simulink model "SWC_HALIN_CDD_type"  (R2021b)
settings: Solver=FixedStepDiscrete  StartTime=0.0  StopTime=10.0  FixedStep=0.005  RelTol=1e-3
values from neighbouring files (symbols this model uses):
  C_TASK_5MS_S = (	C_TICK_TIME_S      	)    [vcu_local_hdr.m]    (also in vcu_local_hdrTA2.m)
  DIDLen_APSFunConfig = uint16(16)    [vcu_local_hdr.m]
  DIDLen_AutoLock = uint16(1)    [vcu_local_hdr.m]
  DIDLen_AutoWipHSpdEN = uint16(1)    [vcu_local_hdr.m]
  DIDLen_DKCKey = uint16(8)    [vcu_local_hdr.m]
  DIDLen_DRLDis = uint16(1)    [vcu_local_hdr.m]
  DIDLen_DynoMode = uint16(1)    [vcu_local_hdr.m]
  DIDLen_FMHTimer = uint16(1)    [vcu_local_hdr.m]
  DIDLen_TireSize = uint16(16)    [vcu_local_hdr.m]
  DIDLen_TurnLampFLThreCurr = uint16(1)    [vcu_local_hdr.m]
  DIDLen_TurnLampFRThreCurr = uint16(1)    [vcu_local_hdr.m]
  DIDLen_TurnLampRLThreCurr = uint16(1)    [vcu_local_hdr.m]
  DIDLen_TurnLampRRThreCurr = uint16(1)    [vcu_local_hdr.m]
  DIDLen_USSConfig = uint16(16)    [vcu_local_hdr.m]
  DIDLen_WipRLSCmdCutFilter = uint16(1)    [vcu_local_hdr.m]
  DIDLen_WipRLSCmdHoldFilter = uint16(1)    [vcu_local_hdr.m]
  DIDLen_XWDMode = uint16(1)    [vcu_local_hdr.m]
  DIDNum_APSFunConfig = uint16(0x0903)    [vcu_local_hdr.m]
  DIDNum_AutoLock = uint16(0x0306)    [vcu_local_hdr.m]
  DIDNum_AutoWipHSpdEN = uint16(0x0308)    [vcu_local_hdr.m]
  DIDNum_DKCKey = uint16(0x0202)    [vcu_local_hdr.m]
  DIDNum_DRLDis = uint16(0x0307)    [vcu_local_hdr.m]
  DIDNum_DynoMode = uint16(0x0203)    [vcu_local_hdr.m]
  DIDNum_FMHTimer = uint16(0x0305)    [vcu_local_hdr.m]
  DIDNum_TireSize = uint16(0x0902)    [vcu_local_hdr.m]
  DIDNum_TurnLampFLThreCurr = uint16(0x0303)    [vcu_local_hdr.m]
  DIDNum_TurnLampFRThreCurr = uint16(0x0301)    [vcu_local_hdr.m]
  DIDNum_TurnLampRLThreCurr = uint16(0x0304)    [vcu_local_hdr.m]
  DIDNum_TurnLampRRThreCurr = uint16(0x0302)    [vcu_local_hdr.m]
  DIDNum_USSConfig = uint16(0x0901)    [vcu_local_hdr.m]
  DIDNum_WipRLSCmdCutFilter = uint16(0x030A)    [vcu_local_hdr.m]
  DIDNum_WipRLSCmdHoldFilter = uint16(0x0309)    [vcu_local_hdr.m]
  DIDNum_XWDMode = uint16(0x0201)    [vcu_local_hdr.m]
  ENUM_DRIVETRAIN_AWD = uint8(  2  )    [vcu_local_hdr.m]
  ENUM_DRIVETRAIN_FWD = uint8(  1  )    [vcu_local_hdr.m]
  ENUM_DRIVETRAIN_RWD = uint8(  0  )    [vcu_local_hdr.m]
  ENUM_REGENLEVEL_LV1 = uint8(  1  )    [vcu_local_hdr.m]
  ENUM_REGENLEVEL_LV2 = uint8(  2  )    [vcu_local_hdr.m]
  ENUM_REGENLEVEL_LV3 = uint8(  3  )    [vcu_local_hdr.m]
  ENUM_REGENLEVEL_LV4 = uint8(  4  )    [vcu_local_hdr.m]
  ENUM_REGENLEVEL_LV5 = uint8(  5  )    [vcu_local_hdr.m]
  ENUM_REGENLEVEL_OPD = uint8(  6  )    [vcu_local_hdr.m]
  ENUM_TPMSSTA_FAT = uint8(  8  )    [vcu_local_hdr.m]
  ENUM_TPMSSTA_LOWBATTERY = uint8(  2  )    [vcu_local_hdr.m]
  ENUM_TPMSSTA_TRIGGER = uint8(  4  )    [vcu_local_hdr.m]
  FALSE = boolean( 0 )    [vcu_local_hdr.m]    (also in vcu_local_hdrTA2.m)
  ONE_INT = uint8(1)    [vcu_local_hdr.m]    (also in vcu_local_hdrTA2.m)
  TRUE = boolean( 1 )    [vcu_local_hdr.m]    (also in vcu_local_hdrTA2.m)
  ZERO_FLOAT = single(0)    [vcu_local_hdr.m]    (also in vcu_local_hdrTA2.m)
  ZERO_INT = uint8(0)    [vcu_local_hdr.m]    (also in vcu_local_hdrTA2.m)
undefined symbols (not defined in the file or in its folder): KHAL_CANBusOffDebounce_s, KHAL_DefaultRegenMode_enum, KHAL_DKCDecryptEnable_flg_ovrdflg, KHAL_DKCDecryptEnable_flg_ovrdval, KHAL_RandomNumberY1_enum, KHAL_RandomNumberY2_enum, KHAL_RandomNumberY_ovrdflg, KHAL_TPMSRESBUTT_flg_ovrdflg, KHAL_TPMSRESBUTT_flg_ovrdval, KINP_ReadVinCode_flg, R_NVMReadCDD_Inner_NVM_ReadOperation
libraries: simulink x112, hcu_lib x23, hdlsllib x8
(part 4 of 7)

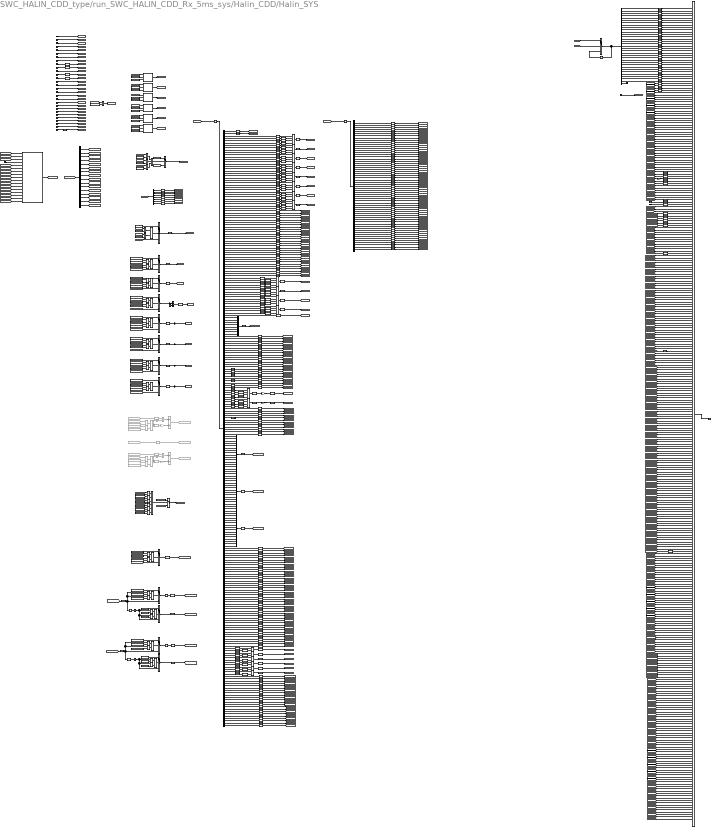
== system SWC_HALIN_CDD_type/run_SWC_HALIN_CDD_Rx_5ms_sys/Halin_CDD/Halin_SYS ==
  note: DID XWD
  note: DID VCUKey
  note: DID BCM
  note: DID APS
  note: CAN bus off debounce
  GetSWID_status : Inport
  GetSWID_data : Inport  Port=2
  VHAL_AnyNMID_flg : Inport  Port=3
  VHAL_CurrentNmState_enum : Inport  Port=4
  VHAL_PwrReq_OTA_enum : Inport  Port=5
  VHAL_AllowMovThd_OTA_enum : Inport  Port=6
  VHAL_EvccAplusPwrUpReq_flg : Inport  Port=7
  VHAL_AcoreReadyToSlp_flg : Inport  Port=8
  VHAL_DidXWDSta_flg : Inport  Port=9
  VHAL_DidXWDData_enum : Inport  Port=10
  HAL_NvmReadData_raw : Inport  Port=11
  VHAL_DIDVCUKeyReadSta_flg : Inport  Port=12
  VHAL_GetDIDVCUKey_enum : Inport  Port=13
  VHAL_NvmProtectSta_flg : Inport  Port=14
  VHAL_AuxBattVolmV_100mV : Inport  Port=15
  VHAL_Pedal1Ref5V_raw : Inport  Port=16
  VHAL_Pedal2Ref5V_raw : Inport  Port=17
  VHAL_NetworkReqCalled_flg : Inport  Port=18
  VHAL_PmicBootReason_enum : Inport  Port=19
  VHAL_WisrBootReason_raw32 : Inport  Port=20
  BHAL_DIDGetData_raw : Inport  Port=21
  VHAL_AcoreRebootCmd_raw : Inport  Port=22
  VHAL_CAN1BusOff_raw : Inport  Port=23
  VHAL_CAN2BusOff_raw : Inport  Port=24
  VHAL_CAN3BusOff_raw : Inport  Port=25
  VHAL_CAN4BusOff_raw : Inport  Port=26
  VHAL_CAN5BusOff_raw : Inport  Port=27
  VHAL_CAN6BusOff_raw : Inport  Port=28
  u8_TPMSSensorIDRegSta : Inport  Port=29
  VHAL_ResetPedalZeroPosReq_raw : Inport  Port=30
  VHAL_PmicBootPath_raw32 : Inport  Port=31
  AND : Logic  Inputs=6  AllPortsSameDT=off  OutDataTypeStr=boolean
  Add1 : Sum
  Bit Shift : hdlsllib/Logic and Bit Operations/Bit Shift  mode=Shift Right Logical  N=1
  Bit Shift1 : hdlsllib/Logic and Bit Operations/Bit Shift  mode=Shift Right Logical  N=1
  Bitwise AND : simulink/Logic and Bit Operations/Bitwise Operator  logicop=AND  UseBitMask=on  BitMask=bin2dec('1')  BitMaskRealWorld=Stored Integer
  Bitwise AND1 : simulink/Logic and Bit Operations/Bitwise Operator  logicop=AND  UseBitMask=on  BitMask=bin2dec('1111111')  BitMaskRealWorld=Stored Integer
  Bitwise AND2 : simulink/Logic and Bit Operations/Bitwise Operator  logicop=AND  UseBitMask=on  BitMask=bin2dec('1')  BitMaskRealWorld=Stored Integer
  Bitwise AND3 : simulink/Logic and Bit Operations/Bitwise Operator  logicop=AND  UseBitMask=on  BitMask=bin2dec('1111111')  BitMaskRealWorld=Stored Integer
  Bitwise OR{1..14} (14 alike) : simulink/Logic and Bit Operations/Bitwise Operator  logicop=OR  UseBitMask=off  NumInputPorts=4  BitMask=bin2dec('00000000000000000000')  BitMaskRealWorld=Stored Integer
  Bitwise OR{15..20} (6 alike) : simulink/Logic and Bit Operations/Bitwise Operator  logicop=OR  UseBitMask=off  NumInputPorts=2  BitMask=bin2dec('00000000000000000000')  BitMaskRealWorld=Stored Integer
  Bus Creator : BusCreator  Inputs=349  OutDataTypeStr=Bus: BHAL_SYS_outputs  NonVirtualBus=on
  Bus Selector : BusSelector  OutputSignals=VHAL_DIDGetXWDMode_raw8,VHAL_DIDGetDKCKey_raw8,VHAL_DIDGetDynoMode_raw8,VHAL_DIDGetTurnLampFRThreCurr_raw8,VHAL_DIDGetTurnLampRRThreCurr_raw8,VHAL_DIDGetTurnLampFLThreCurr_raw8,VHAL_DIDGetTurnLampRLThreCurr_raw8,VHAL_DIDGetFMHTimer_raw8,VHAL_DIDGetAutoLock_raw8,VHAL_DIDGetDRLDis_raw8,VHAL_DIDGetAutoWipHSpdEN_raw8,VHAL_DIDGetWipRLSCmdHoldFilter_raw8,VHAL_DIDGetWipRLSCmdCutFilter_raw8,VHAL_DIDGetUSSConfig_raw8,VHAL_DIDGetTireSize_raw8,VHAL_DIDGetAPSFunConfig_raw8
  Constant{,2..3,10..11,14..15,17,23,26,33,43,47,50,53} (15 alike) : Constant  Value=ZERO_INT
  Constant{1,22,25,41} (4 alike) : Constant  Value=ONE_INT
  Constant12 : Constant  Value=10  OutDataTypeStr=uint8
  Constant{9,13,19..20,28,51,54} (7 alike) : Constant  Value=254  OutDataTypeStr=uint8
  Constant16 : Constant  Value=40  OutDataTypeStr=uint8
  Constant18 : Constant  Value=40  OutDataTypeStr=uint8
  Constant{21,24,42,52,55} (5 alike) : Constant  Value=ZERO_INT  OutDataTypeStr=uint8
  Constant27 : Constant  Value=6  OutDataTypeStr=uint8
  Constant29 : Constant  Commented=on  Value=ONE_INT
  Constant30 : Constant  Commented=on  Value=ZERO_INT
  Constant31 : Constant  Commented=on  Value=ONE_INT
  Constant32 : Constant  Commented=on  Value=ZERO_INT
  Constant34 : Constant  Value=ENUM_REGENLEVEL_LV1
  Constant35 : Constant  Value=ENUM_REGENLEVEL_LV2
  Constant36 : Constant  Value=ENUM_REGENLEVEL_LV3
  Constant37 : Constant  Value=ENUM_REGENLEVEL_LV4
  Constant38 : Constant  Value=ENUM_REGENLEVEL_LV5
  Constant39 : Constant  Value=ENUM_REGENLEVEL_OPD
  Constant4 : Constant  Value=10  OutDataTypeStr=uint8
  Constant40 : Constant  Value=KHAL_DefaultRegenMode_enum
  Constant44 : Constant  Value=126  OutDataTypeStr=uint8
  Constant45 : Constant  Value=10
  Constant46 : Constant  Value=2  OutDataTypeStr=uint8
  Constant48 : Constant  Value=126  OutDataTypeStr=uint8
  Constant49 : Constant  Value=5  OutDataTypeStr=uint8
  Constant5 : Constant  Value=ENUM_DRIVETRAIN_FWD
  Constant{56,58,60,62,64,66} (6 alike) : Constant  Value=C_TASK_5MS_S  OutDataTypeStr=single
  Constant{57,59,61,63,65,67} (6 alike) : Constant  Value=KHAL_CANBusOffDebounce_s  OutDataTypeStr=single
  Constant6 : Constant  Value=ENUM_DRIVETRAIN_RWD
  Constant7 : Constant  Value=ENUM_DRIVETRAIN_AWD
  Constant8 : Constant  Value=ENUM_DRIVETRAIN_RWD
  DIDGet_List : Subsystem
  Data Type Conversion{,3..30,33..44,49..55,98..104,106..107,109,112..128,130..135,139..141,143,164,187,190..195,208..210,212..253,255,273..282,285..286,288..293,296..297,299..358,360..363,814..822} (232 alike) : DataTypeConversion  OutDataTypeStr=uint8
  Data Type Conversion{1..2,31..32,45..48,56..57,105,108,110..111,129,136..138,142,180..185,188..189,200..201,211,283..284,287,294,298,359,823} (37 alike) : DataTypeConversion  OutDataTypeStr=boolean
  Data Type Conversion{58..97,144..163,169..178,186,295} (72 alike) : DataTypeConversion  OutDataTypeStr=uint32
  Data Type Conversion{165..166,168,179,196..199,202} (9 alike) : DataTypeConversion  OutDataTypeStr=single
  Data Type Conversion{167,254,256..272} (19 alike) : DataTypeConversion  OutDataTypeStr=uint16
  Data Type Conversion{203..207} (5 alike) : DataTypeConversion  Commented=on  OutDataTypeStr=uint8
  Demux : Demux  Outputs=33
  Demux1 : Demux  Outputs=256
  Demux2 : Demux  Outputs=8
  Demux3 : Demux  Outputs=61
  Equal{1..5,24..25,28..31} (11 alike) : RelationalOperator  Operator=~=  OutDataTypeStr=boolean  RndMeth=Simplest
  Equal{6,8,10,12,14,16,18,26,32,34,36,38} (12 alike) : RelationalOperator  Operator=>  OutDataTypeStr=boolean  RndMeth=Simplest
  Equal{7,9,11,13,15,17,19,27,33,35,37,39} (12 alike) : RelationalOperator  Operator=<  OutDataTypeStr=boolean  RndMeth=Simplest
  Equal{20..23} (4 alike) : RelationalOperator  Commented=on  Operator=~=  OutDataTypeStr=boolean  RndMeth=Simplest
  FlashAPMDoorControlSta : Subsystem
  FlashCountAlarm_Verify : Subsystem
  FlashFuelDoorPos_Verify : Subsystem
  FlashIVIPTGUSStaSW_Verify : Subsystem
  FlashMFRDNBrightReq_Verify : Subsystem
  FlashMFSWTri_Verify : Subsystem
  FlashMirrorFlodPos_Verify : Subsystem
  FlashWiperFixMode_Verify : Subsystem
  From113 : From  Commented=on  GotoTag=VHAL_DIDGetUSSConfig_raw8
  From114 : From  Commented=on  GotoTag=VHAL_DIDGetTireSize_raw8
  From115 : From  Commented=on  GotoTag=VHAL_DIDGetAPSFunConfig_raw8
  From116 : From  Commented=on  GotoTag=VHAL_DIDGetUSSConfig_raw8
  From117 : From  Commented=on  GotoTag=VHAL_DIDGetUSSConfig_raw8
  From118 : From  Commented=on  GotoTag=VHAL_DIDGetAPSFunConfig_raw8
  From119 : From  Commented=on  GotoTag=VHAL_DIDGetAPSFunConfig_raw8
  Gain2 : Gain  Gain=100
  Gain3 : Gain  Gain=5
  Gain{4..7} (4 alike) : Gain  Gain=10
  Gain8 : Gain  Commented=on  Gain=0xFF  OutDataTypeStr=uint8
  Gain9 : Gain  Commented=on  Gain=0xFF  OutDataTypeStr=uint8
  Goto140 : Goto  Commented=on  GotoTag=VHAL_USSConfig_raw8
  Goto142 : Goto  Commented=on  GotoTag=VHAL_TireSize_raw8
  Goto143 : Goto  Commented=on  GotoTag=VHAL_APSFunConfig_raw8
  Ground : Ground
  Ground1 : Ground
  LatchedFlg{,1..5} (6 alike) : hcu_lib/Basic_Blocks/LatchedFlg
  Logical Operator : Logic  Inputs=3  AllPortsSameDT=off  OutDataTypeStr=boolean
  Logical Operator1 : Logic  AllPortsSameDT=off  OutDataTypeStr=boolean
  Logical Operator{2..13} (12 alike) : Logic  Operator=OR  AllPortsSameDT=off  OutDataTypeStr=boolean
  Multiply1 : Gain  Gain=1/10000
  Multiply2 : Gain  Gain=1/10000
  Mux : Mux  Inputs=8
  Mux1 : Mux  Inputs=16
  Mux2 : Mux  Inputs=16
  Mux3 : Mux  Inputs=16
  NOT : Logic  Commented=on  Operator=NOT  AllPortsSameDT=off  OutDataTypeStr=boolean
  NOT1 : Logic  Commented=on  Operator=NOT  AllPortsSameDT=off  OutDataTypeStr=boolean
  NotEqual : RelationalOperator  Operator=~=  OutDataTypeStr=boolean  RndMeth=Simplest
  OR : Logic  Commented=on  AllPortsSameDT=off  OutDataTypeStr=boolean
  OR1 : Logic  Commented=on  AllPortsSameDT=off  OutDataTypeStr=boolean
  Product : Product  Commented=on
  Product1 : Product  Commented=on
  Selector1 : Selector  InputPortWidth=1024  IndexOptions=Index vector (dialog)  Indices=[1:256]  OutputSizes=1
  Selector2 : Selector  InputPortWidth=1024  IndexOptions=Index vector (dialog)  Indices=[257:317]  OutputSizes=1
  Shift Arithmetic{1,6,9,12,16,21,25,28..29,32,35..37,40,43..48} (20 alike) : ArithShift  BitShiftNumber=8  BitShiftDirection=Left
  Shift Arithmetic{2..3,7,10,13..14,17..18,22,26,30,33,38,41} (14 alike) : ArithShift  BitShiftNumber=16  BitShiftDirection=Left
  Shift Arithmetic{4..5,8,11,15,19..20,23..24,27,31,34,39,42} (14 alike) : ArithShift  BitShiftNumber=24  BitShiftDirection=Left
  Sum : Sum  Commented=on
  Sum1 : Sum  Commented=on
  Switch{,1..15} (16 alike) : Switch  Criteria=u2 ~= 0
  Terminator3 : Terminator
  Unit Delay1 : UnitDelay  SampleTime=-1  HasFrameUpgradeWarning=on
  BHAL_SYS_outputs : Outport  OutDataTypeStr=Bus:BHAL_SYS_outputs
  wires:
  Data Type Conversion49/1 -> [VHAL_RFWheelPSW_raw8]  "VHAL_RFWheelPSW_raw8"
  Demux1/36 -> Data Type Conversion46/1
  Data Type Conversion91/1 -> Shift Arithmetic28/1
  Shift Arithmetic29/1 -> Bitwise OR5/2
  Shift Arithmetic14/1 -> Bitwise OR7/3
  Data Type Conversion73/1 -> Bitwise OR7/1
  Demux/1 -> Data Type Conversion/1
  Data Type Conversion86/1 -> Bitwise OR10/1
  Demux1/39 -> Data Type Conversion51/1
  Demux1/23 -> Data Type Conversion82/1
  Data Type Conversion71/1 -> Shift Arithmetic33/1
  Data Type Conversion48/1 -> [VHAL_RRSensorFail_flg]  "VHAL_RRSensorFail_flg"
  Data Type Conversion11/1 -> Bus Creator/9  "VHAL_Minor2_cnt"
  Data Type Conversion90/1 -> Bitwise OR11/1
  Shift Arithmetic18/1 -> Bitwise OR11/3
  [VHAL_EvccAplusPwrUpReq_flg] -> Data Type Conversion32/1
  Demux1/31 -> Data Type Conversion90/1
  Shift Arithmetic26/1 -> Bitwise OR10/3
  Shift Arithmetic32/1 -> Bitwise OR6/2
  Shift Arithmetic15/1 -> Bitwise OR7/4
  Demux1/30 -> Data Type Conversion89/1
  Data Type Conversion16/1 -> Bus Creator/14  "VHAL_Variation_cnt"
  Data Type Conversion53/1 -> [VHAL_RFPindi_enum]  "VHAL_RFPindi_enum"
  Data Type Conversion95/1 -> [VHAL_FlashRFID_raw]  "VHAL_FlashRFID_raw"
  Demux1/7 -> Data Type Conversion65/1
  Ground/1 -> [VHAL_ReadFlashCorrect_flg]  "VHAL_ReadFlashCorrect_flg"
  Data Type Conversion92/1 -> Shift Arithmetic18/1
  Shift Arithmetic17/1 -> Bitwise OR8/3
  Shift Arithmetic16/1 -> Bitwise OR8/2
  Data Type Conversion54/1 -> [VHAL_FlashAntitheft_enum]  "VHAL_FlashAntitheft_enum"
  Shift Arithmetic22/1 -> Bitwise OR9/3
  Demux1/35 -> Data Type Conversion45/1
  Data Type Conversion78/1 -> [VHAL_FlashChkRFID_raw]  "VHAL_FlashChkRFID_raw"
  Shift Arithmetic21/1 -> Bitwise OR9/2
  Demux1/43 -> Data Type Conversion36/1
  Demux1/25 -> Data Type Conversion84/1
  Demux1/44 -> Data Type Conversion53/1
  Bus Creator/1 -> BHAL_SYS_outputs/1
  Demux1/45 -> Data Type Conversion35/1
  Demux1/14 -> Data Type Conversion72/1
  Demux1/29 -> Data Type Conversion88/1
  Demux1/24 -> Data Type Conversion83/1
  Data Type Conversion35/1 -> [VHAL_LRPindi_enum]  "VHAL_LRPindi_enum"
  Demux1/50 -> Data Type Conversion41/1
  GetSWID_status/1 -> [SYSOut]
  Data Type Conversion37/1 -> [VHAL_RRPindi_enum]  "VHAL_RRPindi_enum"
  Demux1/27 -> Data Type Conversion86/1
  Demux1/6 -> Data Type Conversion64/1
  Demux1/3 -> Data Type Conversion59/1
  Data Type Conversion41/1 -> [VHAL_RRP20_raw8]  "VHAL_RRP20_raw8"
  Constant8/1 -> Switch3/1
  Data Type Conversion70/1 -> Shift Arithmetic32/1
  [VHAL_DIDGetXWDMode_raw8] -> Equal1/1
  Data Type Conversion64/1 -> Shift Arithmetic24/1
  Demux1/9 -> Data Type Conversion67/1
  Shift Arithmetic30/1 -> Bitwise OR5/3
  Bitwise OR10/1 -> Data Type Conversion96/1
  Equal2/1 -> Logical Operator/2
  Equal1/1 -> Logical Operator/1
  Switch3/1 -> [VHAL_DrivetrainSelect_enum]  "VHAL_DrivetrainSelect_enum"
  Data Type Conversion45/1 -> [VHAL_LFSensorFail_flg]  "VHAL_LFSensorFail_flg"
  Data Type Conversion6/1 -> Bus Creator/4  "VHAL_ECU1_cnt"
  Demux/8 -> Data Type Conversion10/1
  Demux1/32 -> Data Type Conversion91/1
  Switch1/1 -> Demux/1, Unit Delay1/1
  Demux/3 -> Data Type Conversion5/1
  Data Type Conversion14/1 -> Bus Creator/12  "VHAL_Country1_cnt"
  Data Type Conversion13/1 -> Bus Creator/11  "VHAL_Patch2_cnt"
  Demux1/46 -> Data Type Conversion37/1
  Demux/11 -> Data Type Conversion13/1
  Demux/14 -> Data Type Conversion16/1
  Data Type Conversion8/1 -> Bus Creator/6  "VHAL_Major1_cnt"
  Data Type Conversion9/1 -> Bus Creator/7  "VHAL_Major2_cnt"
  Demux/13 -> Data Type Conversion15/1
  Shift Arithmetic19/1 -> Bitwise OR11/4
  Demux1/2 -> Data Type Conversion55/1
  Data Type Conversion108/1 -> [VHAL_DIDVCUKeyReadSta_flg]  "VHAL_DIDVCUKeyReadSta_flg"
  Data Type Conversion38/1 -> [VHAL_RFP20_raw8]  "VHAL_RFP20_raw8"
  [VHAL_AcoreReadyToSlp_flg] -> Data Type Conversion1/1
  Demux2/2 -> Data Type Conversion113/1
  Data Type Conversion74/1 -> Shift Arithmetic35/1
  Demux2/5 -> Data Type Conversion116/1
  [VHAL_DIDGetXWDMode_raw8] -> Equal3/1
  Data Type Conversion119/1 -> [VHAL_RandomnumberY_raw8]  "VHAL_RandomnumberY_raw8"
  Demux2/6 -> Data Type Conversion117/1
  Data Type Conversion117/1 -> [VHAL_RandomnumberY_raw6]  "VHAL_RandomnumberY_raw6"
  Demux/9 -> Data Type Conversion11/1
  Data Type Conversion60/1 -> Shift Arithmetic16/1
  Demux1/21 -> Data Type Conversion61/1
  Data Type Conversion114/1 -> [VHAL_RandomnumberY_raw3]  "VHAL_RandomnumberY_raw3"
  Data Type Conversion7/1 -> Bus Creator/5  "VHAL_ECU2_cnt"
  Data Type Conversion116/1 -> [VHAL_RandomnumberY_raw5]  "VHAL_RandomnumberY_raw5"
  Demux2/3 -> Data Type Conversion114/1
  Data Type Conversion115/1 -> [VHAL_RandomnumberY_raw4]  "VHAL_RandomnumberY_raw4"
  Shift Arithmetic25/1 -> Bitwise OR10/2
  Data Type Conversion79/1 -> [VHAL_FlashChkLRID_raw]  "VHAL_FlashChkLRID_raw"
  Data Type Conversion81/1 -> Shift Arithmetic20/1
  Demux/10 -> Data Type Conversion12/1
  Data Type Conversion113/1 -> [VHAL_RandomnumberY_raw2]  "VHAL_RandomnumberY_raw2"
  Data Type Conversion12/1 -> Bus Creator/10  "VHAL_Patch1_cnt"
  Shift Arithmetic20/1 -> Bitwise OR8/4
  Demux1/11 -> Data Type Conversion69/1
  Data Type Conversion10/1 -> Bus Creator/8  "VHAL_Minor1_cnt"
  Data Type Conversion84/1 -> Shift Arithmetic22/1
  Demux1/62 -> Data Type Conversion106/1
  Data Type Conversion94/1 -> [VHAL_FlashLFID_raw]  "VHAL_FlashLFID_raw"
  Demux1/48 -> Data Type Conversion38/1
  Data Type Conversion98/1 -> [VHAL_RFWheelTemp_C]  "VHAL_RFWheelTemp_C"
  Shift Arithmetic12/1 -> Bitwise OR4/2
  Data Type Conversion83/1 -> Shift Arithmetic21/1
  Demux1/49 -> Data Type Conversion39/1
  Demux1/13 -> Data Type Conversion71/1
  Data Type Conversion69/1 -> Bitwise OR6/1
  Demux1/61 -> Data Type Conversion105/1
  Demux1/60 -> Data Type Conversion103/1
  Data Type Conversion104/1 -> [VHAL_Flashchkdatavalid_enum]  "VHAL_Flashchkdatavalid_enum"
  Demux1/59 -> Data Type Conversion104/1
  Bitwise OR7/1 -> Data Type Conversion80/1
  Data Type Conversion103/1 -> [VHAL_Flashdatavalid_enum]  "VHAL_Flashdatavalid_enum"
  Shift Arithmetic23/1 -> Bitwise OR9/4
  Demux1/58 -> Data Type Conversion101/1
  Demux1/20 -> Data Type Conversion60/1
  Data Type Conversion99/1 -> [VHAL_LRWheelTemp_C]  "VHAL_LRWheelTemp_C"
  Demux1/54 -> Data Type Conversion44/1
  Demux/12 -> Data Type Conversion14/1
  Data Type Conversion82/1 -> Bitwise OR9/1
  Demux1/53 -> Data Type Conversion42/1
  Demux1/17 -> Data Type Conversion75/1
  Data Type Conversion96/1 -> [VHAL_FlashLRID_raw]  "VHAL_FlashLRID_raw"
  Demux1/8 -> Data Type Conversion66/1
  Demux1/37 -> Data Type Conversion47/1
  Demux1/34 -> Data Type Conversion93/1
  Demux1/10 -> Data Type Conversion68/1
  Data Type Conversion66/1 -> Shift Arithmetic29/1
  Shift Arithmetic24/1 -> Bitwise OR4/4
  Data Type Conversion15/1 -> Bus Creator/13  "VHAL_Country2_cnt"
  Data Type Conversion50/1 -> [VHAL_LRWheelPSW_raw8]  "VHAL_LRWheelPSW_raw8"
  Data Type Conversion61/1 -> Shift Arithmetic17/1
  Demux/5 -> Data Type Conversion7/1
  Bitwise OR9/1 -> Data Type Conversion95/1
  Data Type Conversion40/1 -> [VHAL_LFP20_raw8]  "VHAL_LFP20_raw8"
  Data Type Conversion112/1 -> [VHAL_RandomnumberY_raw1]  "VHAL_RandomnumberY_raw1"
  Data Type Conversion46/1 -> [VHAL_RFSensorFail_flg]  "VHAL_RFSensorFail_flg"
  Data Type Conversion88/1 -> Shift Arithmetic26/1
  Data Type Conversion67/1 -> Shift Arithmetic30/1
  Data Type Conversion87/1 -> Shift Arithmetic25/1
  Demux1/1 -> Data Type Conversion54/1
  Data Type Conversion127/1 -> [VHAL_FlashAirIntenZone1M_enum]  "VHAL_FlashAirIntenZone1M_enum"
  Demux1/33 -> Data Type Conversion92/1
  Data Type Conversion106/1 -> [VHAL_unlearnSfailvalid_enum]  "VHAL_unlearnSfailvalid_enum"
  Demux1/52 -> Data Type Conversion102/1
  Demux2/1 -> Data Type Conversion112/1
  Data Type Conversion63/1 -> Shift Arithmetic13/1
  Data Type Conversion59/1 -> Bitwise OR4/1
  Demux1/93 -> Data Type Conversion128/1
  Data Type Conversion93/1 -> Shift Arithmetic19/1
  Bitwise OR11/1 -> Data Type Conversion97/1
  VHAL_DIDVCUKeyReadSta_flg/1 -> Data Type Conversion108/1
  Bitwise OR5/1 -> Data Type Conversion78/1
  Data Type Conversion43/1 -> [VHAL_LFWheelPress_raw8]  "VHAL_LFWheelPress_raw8"
  Data Type Conversion62/1 -> Shift Arithmetic12/1
  Demux1/40 -> Data Type Conversion49/1
  Demux1/47 -> Data Type Conversion40/1
  Demux/2 -> Data Type Conversion4/1
  Shift Arithmetic28/1 -> Bitwise OR11/2
  Data Type Conversion128/1 -> [VHAL_FlashFaceM_enum]  "VHAL_FlashFaceM_enum"
  Demux1/57 -> Data Type Conversion99/1
  Demux1/94 -> Data Type Conversion126/1
  Demux1/55 -> Data Type Conversion100/1
  Shift Arithmetic34/1 -> Bitwise OR6/4
  [VHAL_DIDGetDKCKey_raw8] -> Demux2/1
  Demux1/63 -> Data Type Conversion107/1
  Data Type Conversion44/1 -> [VHAL_RRWheelPress_raw8]  "VHAL_RRWheelPress_raw8"
  Demux1/91 -> Data Type Conversion123/1
  Data Type Conversion4/1 -> Bus Creator/2  "VHAL_CarModel2_cnt"
  Data Type Conversion100/1 -> [VHAL_LFWheelTemp_C]  "VHAL_LFWheelTemp_C"
  Data Type Conversion36/1 -> [VHAL_LFPindi_enum]  "VHAL_LFPindi_enum"
  Data Type Conversion76/1 -> Shift Arithmetic15/1
  [VHAL_PwrReq_OTA_enum] -> Data Type Conversion29/1
  Data Type Conversion55/1 -> [VHAL_DIDFlashXWDMode_raw8]  "VHAL_FlashDrivetrain_enum"
  Demux1/42 -> Data Type Conversion52/1
  Data Type Conversion121/1 -> [VHAL_FlashACModeSet123_enum]  "VHAL_FlashACModeSet123_enum"
  Data Type Conversion89/1 -> Shift Arithmetic27/1
  Data Type Conversion72/1 -> Shift Arithmetic34/1
  Data Type Conversion97/1 -> [VHAL_FlashRRID_raw]  "VHAL_FlashRRID_raw"
  Constant6/1 -> Equal2/2
  VHAL_GetDIDVCUKey_enum/1 -> Data Type Conversion109/1
  Data Type Conversion118/1 -> [VHAL_RandomnumberY_raw7]  "VHAL_RandomnumberY_raw7"
  Data Type Conversion85/1 -> Shift Arithmetic23/1
  Demux1/15 -> Data Type Conversion73/1
  [SYSbuffer] -> Switch1/1
  [VHAL_DIDGetXWDMode_raw8] -> Equal2/1
  Data Type Conversion80/1 -> [VHAL_FlashChkRRID_raw]  "VHAL_FlashChkRRID_raw"
  Data Type Conversion123/1 -> [VHAL_FlashFoot_enum]  "VHAL_FlashFoot_enum"
  Demux2/4 -> Data Type Conversion115/1
  Demux1/56 -> Data Type Conversion98/1
  Data Type Conversion132/1 -> [VHAL_Flashfdefog_enum]  "VHAL_Flashfdefog_enum"
  Demux/6 -> Data Type Conversion8/1
  Demux1/5 -> Data Type Conversion63/1
  Data Type Conversion101/1 -> [VHAL_RRWheelTemp_C]  "VHAL_RRWheelTemp_C"
  Data Type Conversion126/1 -> [VHAL_FlashFootM_enum]  "VHAL_FlashFootM_enum"
  Data Type Conversion65/1 -> Bitwise OR5/1
  Demux1/18 -> Data Type Conversion76/1
  Demux/7 -> Data Type Conversion9/1
  Demux/4 -> Data Type Conversion6/1
  Data Type Conversion102/1 -> [VHAL_RFWheelPress_raw8]  "VHAL_RFWheelPress_raw8"
  Data Type Conversion299/1 -> [VHAL_FlashFrost_enum]  "VHAL_FlashFrost_enum"
  [VHAL_DIDGetXWDMode_raw8] -> Switch3/3
  Data Type Conversion68/1 -> Shift Arithmetic31/1
  [SYSOut] -> Switch1/2
  Demux2/7 -> Data Type Conversion118/1
  Unit Delay1/1 -> Switch1/3
  Demux1/16 -> Data Type Conversion74/1
  [VHAL_AllowMovThd_OTA_enum] -> Data Type Conversion30/1
  Demux1/92 -> Data Type Conversion299/1
  Demux1/89 -> Data Type Conversion121/1
  Demux1/26 -> Data Type Conversion85/1
  Shift Arithmetic35/1 -> Bitwise OR7/2
  Bitwise OR4/1 -> Data Type Conversion77/1
  Demux1/100 -> Data Type Conversion132/1
  Logical Operator/1 -> Switch3/2
  Shift Arithmetic33/1 -> Bitwise OR6/3
  Demux1/96 -> Data Type Conversion129/1
  Data Type Conversion5/1 -> Bus Creator/3  "VHAL_CarModel3_cnt"
  Demux1/99 -> Data Type Conversion127/1
  Demux1/90 -> Data Type Conversion122/1
  Data Type Conversion52/1 -> [VHAL_RRWheelPSW_raw8]  "VHAL_RRWheelPSW_raw8"
  Demux1/51 -> Data Type Conversion43/1
  Shift Arithmetic31/1 -> Bitwise OR5/4
  Data Type Conversion131/1 -> [VHAL_FlashRecAutoFlg_enum]  "VHAL_FlashRecAutoFlg_enum"
  Bitwise OR8/1 -> Data Type Conversion94/1
  Data Type Conversion129/1 -> [VHAL_FlashACForceOFF_flg]  "VHAL_FlashACForceOFF_flg"
  Selector1/1 -> Demux1/1
  Data Type Conversion39/1 -> [VHAL_LRP20_raw8]  "VHAL_LRP20_raw8"
  Mux/1 -> Data Type Conversion120/1
  Data Type Conversion47/1 -> [VHAL_LRSensorFail_flg]  "VHAL_LRSensorFail_flg"
  Data Type Conversion42/1 -> [VHAL_LRWheelPress_raw8]  "VHAL_LRWheelPress_raw8"
  Demux1/38 -> Data Type Conversion48/1
  Data Type Conversion75/1 -> Shift Arithmetic14/1
  Data Type Conversion105/1 -> [VHAL_unlearnSfali_flg]  "VHAL_unlearnSfali_flg"
  Shift Arithmetic13/1 -> Bitwise OR4/3
  Data Type Conversion107/1 -> [VHAL_Prepresstempvalid_enum]  "VHAL_Prepresstempvalid_enum"
  Data Type Conversion120/1 -> [VHAL_DIDFlashDKCKey_raw8]
  Equal3/1 -> Logical Operator/3
  Bitwise OR6/1 -> Data Type Conversion79/1
  Data Type Conversion58/1 -> Bitwise OR8/1
  Demux1/22 -> Data Type Conversion81/1
  Data Type Conversion130/1 -> [VHAL_FlashsigRecircSt_enum]  "VHAL_FlashsigRecircSt_enum"
  Data Type Conversion51/1 -> [VHAL_LFWheelPSW_raw8]  "VHAL_LFWheelPSW_raw8"
  Data Type Conversion77/1 -> [VHAL_FlashChkLFID_raw]  "VHAL_FlashChkLFID_raw"
  Data Type Conversion109/1 -> [VHAL_GetDIDVCUKey_raw]  "VHAL_GetDIDVCUKey_enum"
  Data Type Conversion/1 -> Bus Creator/1  "VHAL_CarMode1_cnt"
  Demux2/8 -> Data Type Conversion119/1
  Data Type Conversion122/1 -> [VHAL_FlashFace_enum]  "VHAL_FlashFace_enum"
  Shift Arithmetic27/1 -> Bitwise OR10/4
  Constant7/1 -> Equal3/2
  Constant5/1 -> Equal1/2
  Data Type Conversion125/1 -> [VHAL_FlashCCUSyncSts_enum]  "VHAL_FlashCCUSyncSts_enum"
  Demux1/4 -> Data Type Conversion62/1
  Demux1/41 -> Data Type Conversion50/1
  Demux1/12 -> Data Type Conversion70/1
  Demux1/28 -> Data Type Conversion87/1
  Demux1/19 -> Data Type Conversion58/1
  GetSWID_data/1 -> [SYSbuffer]
  VHAL_AcoreReadyToSlp_flg/1 -> [VHAL_AcoreReadyToSlp_flg]
  VHAL_AllowMovThd_OTA_enum/1 -> [VHAL_AllowMovThd_OTA_enum]
  VHAL_EvccAplusPwrUpReq_flg/1 -> [VHAL_EvccAplusPwrUpReq_flg]
  VHAL_PwrReq_OTA_enum/1 -> [VHAL_PwrReq_OTA_enum]
  VHAL_AnyNMID_flg/1 -> [VHAL_AnyNMID_flg]
  VHAL_CurrentNmState_enum/1 -> [VHAL_CurrentNmState_enum]
  Data Type Conversion2/1 -> [VHAL_DidXWDSta_flg]  "VHAL_DidXWDSta_flg"
  VHAL_DidXWDSta_flg/1 -> Data Type Conversion2/1
  Data Type Conversion3/1 -> [VHAL_DidXWDData_enum]  "VHAL_DidXWDData_enum"
  VHAL_DidXWDData_enum/1 -> Data Type Conversion3/1
  HAL_NvmReadData_raw/1 -> [HAL_NvmReadData_raw]
  [HAL_NvmReadData_raw] -> Selector1/1
  [VHAL_CurrentNmState_enum] -> Data Type Conversion33/1
  [VHAL_AnyNMID_flg] -> Data Type Conversion31/1
  Data Type Conversion134/1 -> [VHAL_FlashsigSetTempZon2StM_C]  "VHAL_FlashsigSetTempZon2StM_C"
  FlashMFSWTri_Verify/1(Out1) -> Data Type Conversion136/1
  Data Type Conversion142/1 -> [VHAL_FlashWiperFixMode_flg]  "VHAL_FlashWiperFixMode_flg"
  FlashWiperFixMode_Verify/1(Out1) -> Data Type Conversion142/1
  FlashFuelDoorPos_Verify/1(Out1) -> Data Type Conversion138/1
  FlashIVIPTGUSStaSW_Verify/1(Out1) -> Data Type Conversion143/1
  Data Type Conversion135/1 -> [VHAL_FlashCountAlarm_enum]  "VHAL_FlashCountAlarm_enum"
  FlashMFRDNBrightReq_Verify/1(Out1) -> Data Type Conversion140/1
  Data Type Conversion140/1 -> [VHAL_FlashMFRDNBrightReq_pct]  "VHAL_FlashMFRDNBrightReq_pct"
  Data Type Conversion138/1 -> [VHAL_FlashFuelDoorPos_flg]  "VHAL_FlashFuelDoorPos_flg"
  Demux1/102 -> Data Type Conversion134/1
  Data Type Conversion133/1 -> [VHAL_FlashsigSetTempZon1St_C]  "VHAL_FlashsigSetTempZon1St_C"
  Data Type Conversion136/1 -> [VHAL_FlashMFSWTri_flg]  "VHAL_FlashMFSWTri_flg"
  FlashMirrorFlodPos_Verify/1(Out1) -> Data Type Conversion137/1
  Demux1/101 -> Data Type Conversion133/1
  Data Type Conversion137/1 -> [VHAL_FlashMirrorFlodPos_flg]  "VHAL_FlashMirrorFlodPos_flg"
  FlashCountAlarm_Verify/1(Out1) -> Data Type Conversion135/1
  Data Type Conversion150/1 -> Shift Arithmetic7/1
  Data Type Conversion156/1 -> Bitwise OR12/1
  Data Type Conversion147/1 -> Shift Arithmetic5/1
  Data Type Conversion151/1 -> Shift Arithmetic8/1
  Data Type Conversion161/1 -> [VHAL_FlashS2ID_raw]  "VHAL_FlashS2ID_raw"
  Demux1/66 -> Data Type Conversion146/1
  Demux1/64 -> Data Type Conversion144/1
  Data Type Conversion158/1 -> Shift Arithmetic3/1
  Demux1/79 -> Data Type Conversion159/1
  Data Type Conversion153/1 -> Shift Arithmetic9/1
  Shift Arithmetic8/1 -> Bitwise OR2/4
  Data Type Conversion144/1 -> Bitwise OR1/1
  Data Type Conversion154/1 -> Shift Arithmetic10/1
  Data Type Conversion159/1 -> Shift Arithmetic4/1
  Shift Arithmetic4/1 -> Bitwise OR12/4
  Demux1/70 -> Data Type Conversion150/1
  Demux1/71 -> Data Type Conversion151/1
  Data Type Conversion148/1 -> Bitwise OR2/1
  Demux1/80 -> Data Type Conversion164/1
  Shift Arithmetic5/1 -> Bitwise OR1/4
  Shift Arithmetic36/1 -> Bitwise OR12/2
  Demux1/68 -> Data Type Conversion148/1
  Shift Arithmetic1/1 -> Bitwise OR1/2
  Demux1/78 -> Data Type Conversion158/1
  Data Type Conversion146/1 -> Shift Arithmetic2/1
  Demux1/67 -> Data Type Conversion147/1
  Shift Arithmetic3/1 -> Bitwise OR12/3
  Data Type Conversion163/1 -> [VHAL_FlashS4ID_raw]  "VHAL_FlashS4ID_raw"
  Demux1/72 -> Data Type Conversion152/1
  Data Type Conversion155/1 -> Shift Arithmetic11/1
  Data Type Conversion160/1 -> [VHAL_FlashS1ID_raw]  "VHAL_FlashS1ID_raw"
  Demux1/69 -> Data Type Conversion149/1
  Bitwise OR12/1 -> Data Type Conversion163/1
  Data Type Conversion157/1 -> Shift Arithmetic36/1
  Bitwise OR1/1 -> Data Type Conversion160/1
  Shift Arithmetic10/1 -> Bitwise OR3/3
  Bitwise OR3/1 -> Data Type Conversion162/1
  Data Type Conversion162/1 -> [VHAL_FlashS3ID_raw]  "VHAL_FlashS3ID_raw"
  Shift Arithmetic7/1 -> Bitwise OR2/3
  Demux1/75 -> Data Type Conversion155/1
  Demux1/74 -> Data Type Conversion154/1
  Shift Arithmetic2/1 -> Bitwise OR1/3
  Data Type Conversion164/1 -> [VHAL_FlashIDvaild_enum]  "VHAL_FlashIDvalid_enum"
  Bitwise OR2/1 -> Data Type Conversion161/1
  Demux1/65 -> Data Type Conversion145/1
  Data Type Conversion149/1 -> Shift Arithmetic6/1
  Data Type Conversion145/1 -> Shift Arithmetic1/1
  Shift Arithmetic6/1 -> Bitwise OR2/2
  Shift Arithmetic11/1 -> Bitwise OR3/4
  Demux1/76 -> Data Type Conversion156/1
  Demux1/73 -> Data Type Conversion153/1
  Data Type Conversion152/1 -> Bitwise OR3/1
  Demux1/77 -> Data Type Conversion157/1
  Shift Arithmetic9/1 -> Bitwise OR3/2
  Demux1/81 -> Mux/1
  Demux1/82 -> Mux/2
  Demux1/83 -> Mux/3
  Demux1/84 -> Mux/4
  Demux1/85 -> Mux/5
  Demux1/86 -> Mux/6
  Demux1/87 -> Mux/7
  Demux1/88 -> Mux/8
  Demux1/95 -> Data Type Conversion125/1
  Demux1/97 -> Data Type Conversion130/1
  Demux1/98 -> Data Type Conversion131/1
  Demux1/103 -> FlashCountAlarm_Verify/1(In1)
  Demux1/104 -> FlashMFSWTri_Verify/1(In1)
  Demux1/105 -> FlashMirrorFlodPos_Verify/1(In1)
  Demux1/106 -> FlashFuelDoorPos_Verify/1(In1)
  Demux1/108 -> FlashMFRDNBrightReq_Verify/1(In1)
  Demux1/110 -> FlashWiperFixMode_Verify/1(In1)
  Demux1/111 -> FlashIVIPTGUSStaSW_Verify/1(In1)
  [VHAL_NvmProtectSta_flg] -> Data Type Conversion56/1
  VHAL_NvmProtectSta_flg/1 -> [VHAL_NvmProtectSta_flg]
  [VHAL_Pedal1Ref5V_raw] -> Data Type Conversion165/1
  [VHAL_Pedal2Ref5V_raw] -> Data Type Conversion166/1
  VHAL_AuxBattVolmV_100mV/1 -> [VHAL_AuxBattVolmV_100mV]
  VHAL_Pedal2Ref5V_raw/1 -> [VHAL_Pedal2Ref5V_raw]
  VHAL_Pedal1Ref5V_raw/1 -> [VHAL_Pedal1Ref5V_raw]
  [VHAL_AuxBattVolmV_100mV] -> Gain2/1
  Demux1/117 -> Data Type Conversion175/1
  Demux1/116 -> Data Type Conversion174/1
  Bitwise OR13/1 -> Data Type Conversion173/1
  Data Type Conversion177/1 -> Shift Arithmetic42/1
  Shift Arithmetic38/1 -> Bitwise OR13/3
  Demux1/114 -> Data Type Conversion171/1
  Shift Arithmetic41/1 -> Bitwise OR14/3
  Demux1/119 -> Data Type Conversion177/1
  Multiply2/1 -> Data Type Conversion168/1
  Data Type Conversion178/1 -> Multiply2/1
  Data Type Conversion175/1 -> Shift Arithmetic40/1
  Data Type Conversion173/1 -> Multiply1/1
  Shift Arithmetic42/1 -> Bitwise OR14/4
  Data Type Conversion176/1 -> Shift Arithmetic41/1
  Demux1/113 -> Data Type Conversion170/1
  Bitwise OR14/1 -> Data Type Conversion178/1
  Shift Arithmetic40/1 -> Bitwise OR14/2
  Data Type Conversion170/1 -> Shift Arithmetic37/1
  Data Type Conversion171/1 -> Shift Arithmetic38/1
  Data Type Conversion174/1 -> Bitwise OR14/1
  Data Type Conversion179/1 -> [VHAL_EAPS1MINMem_pct]  "VHAL_EAPS1MINMem_pct"
  Demux1/118 -> Data Type Conversion176/1
  Shift Arithmetic37/1 -> Bitwise OR13/2
  Demux1/115 -> Data Type Conversion172/1
  Demux1/112 -> Data Type Conversion169/1
  Data Type Conversion169/1 -> Bitwise OR13/1
  Shift Arithmetic39/1 -> Bitwise OR13/4
  Multiply1/1 -> Data Type Conversion179/1
  Data Type Conversion172/1 -> Shift Arithmetic39/1
  Data Type Conversion168/1 -> [VHAL_EAPS2MINMem_pct]  "VHAL_EAPS2MINMem_pct"
  Demux1/120 -> Data Type Conversion180/1
  Demux1/121 -> Data Type Conversion181/1
  Demux1/122 -> Data Type Conversion182/1
  Demux1/123 -> Data Type Conversion183/1
  Data Type Conversion180/1 -> [VHAL_FlashHoodSW_flg]  "VHAL_FlashHoodSW_flg"
  Data Type Conversion181/1 -> [VHAL_FlashTailgateSW_flg]  "VHAL_FlashTailgateSW_flg"
  Data Type Conversion182/1 -> [VHAL_FlashCTDLockSW_flg]  "VHAL_FlashCTDLockSW_flg"
  Data Type Conversion183/1 -> [VHAL_FlashTailgateHDSW_flg]  "VHAL_FlashTailgateHDSW_flg"
  VHAL_NetworkReqCalled_flg/1 -> [VHAL_NetworkReqCalled_flg]
  [VHAL_NetworkReqCalled_flg] -> Data Type Conversion184/1
  Gain2/1 -> Data Type Conversion167/1
  VHAL_PmicBootReason_enum/1 -> Data Type Conversion187/1
  VHAL_WisrBootReason_raw32/1 -> Data Type Conversion186/1
  Demux1/124 -> FlashAPMDoorControlSta/1(In1)
  FlashAPMDoorControlSta/1(Out1) -> Data Type Conversion185/1
  Data Type Conversion185/1 -> [VHAL_FlashAPMDoorControlSta_flg]  "VHAL_FlashAPMDoorControlSta_flg"
  BHAL_DIDGetData_raw/1 -> [BHAL_DIDGetData_raw]
  VHAL_AcoreRebootCmd_raw/1 -> [VHAL_AcoreRebootCmd_raw]  "VHAL_AcoreRebootCmd_raw"
  Switch/1 -> Data Type Conversion298/1
  VHAL_CAN1BusOff_raw/1 -> [VHAL_CAN1BusOff_raw]
  VHAL_CAN2BusOff_raw/1 -> [VHAL_CAN2BusOff_raw]
  VHAL_CAN3BusOff_raw/1 -> [VHAL_CAN3BusOff_raw]
  VHAL_CAN4BusOff_raw/1 -> [VHAL_CAN4BusOff_raw]
  VHAL_CAN5BusOff_raw/1 -> [VHAL_CAN5BusOff_raw]
  [VHAL_CAN1BusOff_flg] -> Data Type Conversion57/1
  [VHAL_CAN2BusOff_flg] -> Data Type Conversion110/1
  [VHAL_CAN3BusOff_flg] -> Data Type Conversion188/1
  [VHAL_CAN4BusOff_flg] -> Data Type Conversion111/1
  [VHAL_CAN5BusOff_flg] -> Data Type Conversion189/1
  Constant1/1 -> Equal4/2
  [VHAL_DIDGetDynoMode_raw8] -> Equal4/1
  [VHAL_DIDGetDynoMode_raw8] -> Equal5/1
  Constant2/1 -> Equal5/2
  Equal4/1 -> Logical Operator1/1
  Equal5/1 -> Logical Operator1/2
  Logical Operator1/1 -> Switch/2
  Constant3/1 -> Switch/1
  [VHAL_DIDGetDynoMode_raw8] -> Switch/3
  [VHAL_AcoreRebootCmd_raw] -> NotEqual/1
  Constant/1 -> NotEqual/2
  NotEqual/1 -> [VHAL_AcoreRebootCmd_flg]
  Data Type Conversion202/1 -> [VHAL_DiagFMHT_s]  "VHAL_DiagFMHT_s"
  [VHAL_DIDGetAutoLock_raw8] -> Equal15/1
  Equal10/1 -> Logical Operator4/1
  Switch9/1 -> Gain3/1
  [VHAL_DIDGetTurnLampFRThreCurr_raw8] -> Switch4/3
  Constant20/1 -> Equal10/2
  Gain7/1 -> [VHAL_DiagRRTC_mA]  "VHAL_DiagRRTC_mA"
  [VHAL_DIDGetTurnLampRLThreCurr_raw8] -> Equal10/1
  Equal11/1 -> Logical Operator4/2
  Gain5/1 -> [VHAL_DiagFRTC_mA]  "VHAL_DiagFRTC_mA"
  Gain6/1 -> [VHAL_DiagRLTC_mA]  "VHAL_DiagRLTC_mA"
  Constant45/1 -> Add1/2
  Add1/1 -> Data Type Conversion202/1
  Data Type Conversion201/1 -> [VHAL_DiagDRLOFF_flg]  "VHAL_DiagDRLOFF_flg"
  Logical Operator4/1 -> Switch5/2
  [VHAL_DIDGetTurnLampRLThreCurr_raw8] -> Switch5/3
  Equal19/1 -> Logical Operator8/2
  Equal13/1 -> Logical Operator5/2
  Switch8/1 -> Data Type Conversion201/1
  Gain4/1 -> [VHAL_DiagFLTC_mA]  "VHAL_DiagFLTC_mA"
  Constant28/1 -> Equal18/2
  Switch4/1 -> Data Type Conversion197/1
  Switch2/1 -> Data Type Conversion196/1
  Constant21/1 -> Switch7/1
  Data Type Conversion196/1 -> Gain4/1
  Data Type Conversion197/1 -> Gain5/1
  Gain3/1 -> Add1/1
  Logical Operator7/1 -> Switch8/2
  Equal16/1 -> Logical Operator7/1
  Constant26/1 -> Equal19/2
  [VHAL_DIDGetDRLDis_raw8] -> Equal16/1
  [VHAL_DIDGetFMHTimer_raw8] -> Equal18/1
  Constant16/1 -> Switch6/1
  [VHAL_DIDGetFMHTimer_raw8] -> Equal19/1
  [VHAL_DIDGetFMHTimer_raw8] -> Switch9/3
  Constant23/1 -> Equal17/2
  [VHAL_DIDGetTurnLampFRThreCurr_raw8] -> Equal8/1
  Constant10/1 -> Equal7/2
  Data Type Conversion199/1 -> Gain7/1
  Constant12/1 -> Switch4/1
  [VHAL_DIDGetDRLDis_raw8] -> Equal17/1
  [VHAL_DIDGetDRLDis_raw8] -> Switch8/3
  Equal7/1 -> Logical Operator2/2
  [VHAL_DIDGetAutoLock_raw8] -> Equal14/1
  Equal17/1 -> Logical Operator7/2
  [VHAL_DIDGetTurnLampRLThreCurr_raw8] -> Equal11/1
  Constant25/1 -> Equal16/2
  Data Type Conversion200/1 -> [VHAL_funAuto_flg]  "VHAL_funAuto_flg"
  Switch7/1 -> Data Type Conversion200/1
  Constant17/1 -> Equal15/2
  Switch6/1 -> Data Type Conversion199/1
  Constant27/1 -> Switch9/1
  Switch5/1 -> Data Type Conversion198/1
  Logical Operator3/1 -> Switch4/2
  Constant11/1 -> Equal9/2
  Constant14/1 -> Equal11/2
  Constant24/1 -> Switch8/1
  Constant15/1 -> Equal13/2
  Data Type Conversion198/1 -> Gain6/1
  [VHAL_DIDGetTurnLampFLThreCurr_raw8] -> Equal6/1
  [VHAL_DIDGetTurnLampRRThreCurr_raw8] -> Equal12/1
  [VHAL_DIDGetTurnLampRRThreCurr_raw8] -> Equal13/1
  Equal12/1 -> Logical Operator5/1
  Constant13/1 -> Equal8/2
  Equal14/1 -> Logical Operator6/1
  Logical Operator8/1 -> Switch9/2
  Constant22/1 -> Equal14/2
  [VHAL_DIDGetTurnLampFRThreCurr_raw8] -> Equal9/1
  Constant19/1 -> Equal12/2
  Equal8/1 -> Logical Operator3/1
  [VHAL_DIDGetTurnLampFLThreCurr_raw8] -> Switch2/3
  Equal6/1 -> Logical Operator2/1
  Constant18/1 -> Switch5/1
  Logical Operator2/1 -> Switch2/2
  [VHAL_DIDGetTurnLampFLThreCurr_raw8] -> Equal7/1
  Equal9/1 -> Logical Operator3/2
  [VHAL_DIDGetAutoLock_raw8] -> Switch7/3
  Logical Operator6/1 -> Switch7/2
  Equal15/1 -> Logical Operator6/2
  Constant9/1 -> Equal6/2
  [VHAL_DIDGetTurnLampRRThreCurr_raw8] -> Switch6/3
  Logical Operator5/1 -> Switch6/2
  Constant4/1 -> Switch2/1
  Equal18/1 -> Logical Operator8/1
  Demux1/131 -> Data Type Conversion190/1
  Demux1/129 -> Data Type Conversion34/1
  Data Type Conversion34/1 -> [VHAL_DIDFlashTurnLampFRThreCurr_raw8]  "VHAL_DIDFlashTurnLampFRThreCurr_raw8"
  Demux1/130 -> Data Type Conversion192/1
  Demux1/128 -> Data Type Conversion191/1
  Demux1/127 -> Data Type Conversion193/1
  Demux1/126 -> Data Type Conversion195/1
  Data Type Conversion192/1 -> [VHAL_DIDFlashTurnLampRLThreCurr_raw8]  "VHAL_DIDFlashTurnLampRLThreCurr_raw8"
  Data Type Conversion195/1 -> [VHAL_DIDFlashDRLDis_raw8]  "VHAL_DIDFlashDRLDis_raw8"
  Data Type Conversion190/1 -> [VHAL_DIDFlashTurnLampRRThreCurr_raw8]  "VHAL_DIDFlashTurnLampRRThreCurr_raw8"
  Data Type Conversion193/1 -> [VHAL_DIDFlashFMHTimer_raw8]  "VHAL_DIDFlashFMHTimer_raw8"
  Demux1/125 -> Data Type Conversion194/1
  Data Type Conversion191/1 -> [VHAL_DIDFlashTurnLampFLThreCurr_raw8]  "VHAL_DIDFlashTurnLampFLThreCurr_raw8"
  Data Type Conversion194/1 -> [VHAL_DIDFlashAutoLock_raw8]  "VHAL_DIDFlashAutoLock_raw8"
  Equal20/1 -> OR/1
  From113/1 -> Equal20/1
  Constant29/1 -> Equal20/2
  From116/1 -> Equal21/1
  Constant30/1 -> Equal21/2
  Equal21/1 -> OR/2
  Data Type Conversion203/1 -> Gain8/1
  OR/1 -> NOT/1, Data Type Conversion203/1
  NOT/1 -> Product/2
  From117/1 -> Data Type Conversion204/1
  Product/1 -> Sum/1
  Gain8/1 -> Sum/2
  Data Type Conversion204/1 -> Product/1
  Sum/1 -> Goto140/1
  Sum1/1 -> Goto143/1
  Data Type Conversion206/1 -> Product1/1
  Gain9/1 -> Sum1/2
  Product1/1 -> Sum1/1
  From115/1 -> Data Type Conversion206/1
  NOT1/1 -> Product1/2
  OR1/1 -> Data Type Conversion205/1, NOT1/1
  Data Type Conversion205/1 -> Gain9/1
  Equal23/1 -> OR1/2
  Constant32/1 -> Equal23/2
  From119/1 -> Equal23/1
  Constant31/1 -> Equal22/2
  From118/1 -> Equal22/1
  Equal22/1 -> OR1/1
  From114/1 -> Data Type Conversion207/1
  Data Type Conversion207/1 -> Goto142/1
  Demux1/132 -> Mux1/1
  Demux1/133 -> Mux1/2
  Demux1/134 -> Mux1/3
  Demux1/135 -> Mux1/4
  Demux1/136 -> Mux1/5
  Demux1/137 -> Mux1/6
  Demux1/138 -> Mux1/7
  Demux1/139 -> Mux1/8
  Demux1/140 -> Mux1/9
  Demux1/141 -> Mux1/10
  Demux1/142 -> Mux1/11
  Demux1/143 -> Mux1/12
  Demux1/144 -> Mux1/13
  Demux1/145 -> Mux1/14
  Demux1/146 -> Mux1/15
  Demux1/147 -> Mux1/16
  Mux1/1 -> Data Type Conversion208/1
  Data Type Conversion208/1 -> [VHAL_DIDFlashUSSConfig_raw8]  "VHAL_DIDFlashUSSConfig_raw8"
  Mux2/1 -> Data Type Conversion209/1
  Demux1/163 -> Mux2/16
  Demux1/162 -> Mux2/15
  Demux1/161 -> Mux2/14
  Demux1/160 -> Mux2/13
  Demux1/159 -> Mux2/12
  Demux1/158 -> Mux2/11
  Demux1/157 -> Mux2/10
  Demux1/156 -> Mux2/9
  Demux1/155 -> Mux2/8
  Demux1/154 -> Mux2/7
  Demux1/153 -> Mux2/6
  Demux1/152 -> Mux2/5
  Demux1/151 -> Mux2/4
  Demux1/150 -> Mux2/3
  Demux1/149 -> Mux2/2
  Demux1/148 -> Mux2/1
  Demux1/164 -> Mux3/1
  Demux1/165 -> Mux3/2
  Demux1/166 -> Mux3/3
  Demux1/167 -> Mux3/4
  Demux1/168 -> Mux3/5
  Demux1/169 -> Mux3/6
  Demux1/170 -> Mux3/7
  Demux1/171 -> Mux3/8
  Demux1/172 -> Mux3/9
  Demux1/173 -> Mux3/10
  Demux1/174 -> Mux3/11
  Demux1/175 -> Mux3/12
  Demux1/176 -> Mux3/13
  Demux1/177 -> Mux3/14
  Demux1/178 -> Mux3/15
  Demux1/179 -> Mux3/16
  Mux3/1 -> Data Type Conversion210/1
  Data Type Conversion209/1 -> [VHAL_DIDFlashTireSize_raw8]  "VHAL_DIDFlashTireSize_raw8"
  Data Type Conversion210/1 -> [VHAL_DIDFlashAPSFunConfig_raw8]  "VHAL_DIDFlashAPSFunConfig_raw8"
  Demux1/180 -> Data Type Conversion211/1
  Data Type Conversion211/1 -> [VHAL_FlashfUnlockSingle_flg]  "VHAL_FlashfUnlockSingle_flg"
  Demux1/181 -> Data Type Conversion212/1
  Data Type Conversion212/1 -> [VHAL_ReadRegenMode_enum]  "VHAL_ReadRegenMode_enum"
  [VHAL_FlashRegenMode_enum] -> Data Type Conversion213/1
  Equal28/1 -> AND/1
  Constant36/1 -> Equal30/2
  Equal24/1 -> AND/5
  Equal25/1 -> AND/6
  [VHAL_ReadRegenMode_enum] -> Equal31/1
  Equal30/1 -> AND/3
  Equal31/1 -> AND/4
  AND/1 -> Switch10/2
  Constant39/1 -> Equal25/2
  Constant40/1 -> Switch10/1
  Equal29/1 -> AND/2
  [VHAL_ReadRegenMode_enum] -> Equal24/1
  [VHAL_ReadRegenMode_enum] -> Equal25/1
  [VHAL_ReadRegenMode_enum] -> Switch10/3
  [VHAL_ReadRegenMode_enum] -> Equal29/1
  Constant38/1 -> Equal24/2
  Constant35/1 -> Equal29/2
  [VHAL_ReadRegenMode_enum] -> Equal30/1
  Constant34/1 -> Equal28/2
  [VHAL_ReadRegenMode_enum] -> Equal28/1
  Switch10/1 -> [VHAL_FlashRegenMode_enum]
  Constant37/1 -> Equal31/2
  Data Type Conversion226/1 -> [VHAL_FlashAmbBrightnessSta1_enum]  "VHAL_FlashAmbBrightnessSta1_enum"
  Data Type Conversion228/1 -> [VHAL_FlashAmbBrightnessSta3_enum]  "VHAL_FlashAmbBrightnessSta3_enum"
  Demux1/189 -> Data Type Conversion221/1
  Demux1/187 -> Data Type Conversion220/1
  Data Type Conversion231/1 -> [VHAL_FlashAmbBrightnessSta7_enum]  "VHAL_FlashAmbBrightnessSta7_enum"
  Demux1/195 -> Data Type Conversion227/1
  Demux1/182 -> Data Type Conversion215/1
  Data Type Conversion230/1 -> [VHAL_FlashAmbBrightnessSta5_enum]  "VHAL_FlashAmbBrightnessSta5_enum"
  Demux1/185 -> Data Type Conversion218/1
  Data Type Conversion225/1 -> [VHAL_FlashAmbColorSta7_enum]  "VHAL_FlashAmbColorSta7_enum"
  Data Type Conversion215/1 -> [VHAL_FlashAmbFunEN_enum]  "VHAL_FlashAmbFunEN_enum"
  Demux1/186 -> Data Type Conversion219/1
  Data Type Conversion220/1 -> [VHAL_FlashAmbODAEN_enum]  "VHAL_FlashAmbODAEN_enum"
  Demux1/193 -> Data Type Conversion225/1
  Data Type Conversion222/1 -> [VHAL_FlashAmbColorSta3_enum]  "VHAL_FlashAmbColorSta3_enum"
  Demux1/199 -> Data Type Conversion231/1
  Data Type Conversion216/1 -> [VHAL_FlashAmbWelEN_enum]  "VHAL_FlashAmbWelEN_enum"
  Data Type Conversion218/1 -> [VHAL_FlashAmbLinkDriSta_enum]  "VHAL_FlashAmbLinkDriSta_enum"
  Demux1/191 -> Data Type Conversion223/1
  Demux1/192 -> Data Type Conversion224/1
  Demux1/194 -> Data Type Conversion226/1
  Demux1/196 -> Data Type Conversion228/1
  Data Type Conversion219/1 -> [VHAL_FlashAmbPwrWarnEN_enum]  "VHAL_FlashAmbPwrWarnEN_enum"
  Data Type Conversion214/1 -> [VHAL_FlashAmbColorSta1_enum]  "VHAL_FlashAmbColorSta1_enum"
  Data Type Conversion221/1 -> [VHAL_FlashAmbColorSta2_enum]  "VHAL_FlashAmbColorSta2_enum"
  Data Type Conversion223/1 -> [VHAL_FlashAmbColorSta4_enum]  "VHAL_FlashAmbColorSta4_enum"
  Demux1/197 -> Data Type Conversion229/1
  Demux1/183 -> Data Type Conversion216/1
  Demux1/190 -> Data Type Conversion222/1
  Data Type Conversion229/1 -> [VHAL_FlashAmbBrightnessSta4_enum]  "VHAL_FlashAmbBrightnessSta4_enum"
  Demux1/184 -> Data Type Conversion217/1
  Data Type Conversion227/1 -> [VHAL_FlashAmbBrightnessSta2_enum]  "VHAL_FlashAmbBrightnessSta2_enum"
  Demux1/188 -> Data Type Conversion214/1
  Demux1/198 -> Data Type Conversion230/1
  Data Type Conversion224/1 -> [VHAL_FlashAmbColorSta5_enum]  "VHAL_FlashAmbColorSta5_enum"
  Data Type Conversion217/1 -> [VHAL_FlashAmbDimEN_enum]  "VHAL_FlashAmbDimEN_enum"
  Data Type Conversion245/1 -> [VHAL_FlashDrEVentZSta_enum]  "VHAL_FlashDrEVentZSta_enum"
  Demux1/204 -> Data Type Conversion244/1
  Demux1/218 -> Data Type Conversion250/1
  Data Type Conversion250/1 -> [VHAL_FlashFGSChSta_enum]  "VHAL_FlashFGSChSta_enum"
  Data Type Conversion232/1 -> [VHAL_FlashTurnSwTSet123_enum]  "VHAL_FlashTurnSwTSet123_enum"
  Demux1/209 -> Data Type Conversion235/1
  Data Type Conversion249/1 -> [VHAL_FlashFGSAirIntSta_enum]  "VHAL_FlashFGSAirIntSta_enum"
  Data Type Conversion233/1 -> [VHAL_FlashTurnSwTSet457_enum]  "VHAL_FlashTurnSwTSet457_enum"
  Data Type Conversion124/1 -> [VHAL_FlashFGSIONSWSta_enum]  "VHAL_FlashFGSIONSWSta_enum"
  Data Type Conversion248/1 -> [VHAL_FlashCREVentZSta_enum]  "VHAL_FlashCREVentZSta_enum"
  Data Type Conversion241/1 -> [VHAL_FlashPsEVentYSta_enum]  "VHAL_FlashPsEVentYSta_enum"
  Demux1/219 -> Data Type Conversion124/1
  Data Type Conversion235/1 -> [VHAL_FlashDrVentEN_enum]  "VHAL_FlashDrVentEN_enum"
  Demux1/212 -> Data Type Conversion239/1
  Demux1/217 -> Data Type Conversion249/1
  Demux1/200 -> Data Type Conversion232/1
  Data Type Conversion244/1 -> [VHAL_FlashDrEVentModeSta_enum]  "VHAL_FlashDrEVentModeSta_enum"
  Demux1/203 -> Data Type Conversion243/1
  Demux1/216 -> Data Type Conversion236/1
  Data Type Conversion242/1 -> [VHAL_FlashCRVentEN_enum]  "VHAL_FlashCRVentEN_enum"
  Data Type Conversion238/1 -> [VHAL_FlashCLVentEN_enum]  "VHAL_FlashCLVentEN_enum"
  Demux1/210 -> Data Type Conversion237/1
  Data Type Conversion240/1 -> [VHAL_FlashPsVentEN_enum]  "VHAL_FlashPsVentEN_enum"
  Data Type Conversion236/1 -> [VHAL_FlashCREVentYSta_enum]  "VHAL_FlashCREVentYSta_enum"
  Demux1/214 -> Data Type Conversion241/1
  Demux1/205 -> Data Type Conversion245/1
  Demux1/202 -> Data Type Conversion234/1
  Data Type Conversion247/1 -> [VHAL_FlashPsEVentZSta_enum]  "VHAL_FlashPsEVentZSta_enum"
  Data Type Conversion237/1 -> [VHAL_FlashDrEVentYSta_enum]  "VHAL_FlashDrEVentYSta_enum"
  Data Type Conversion243/1 -> [VHAL_FlashPsEVentModeSta_enum]  "VHAL_FlashPsEVentModeSta_enum"
  Demux1/215 -> Data Type Conversion242/1
  Data Type Conversion234/1 -> [VHAL_FlashAirIntZ3Sta_enum]  "VHAL_FlashAirIntZ3Sta_enum"
  Demux1/211 -> Data Type Conversion238/1
  Demux1/206 -> Data Type Conversion246/1
  Data Type Conversion239/1 -> [VHAL_FlashCLEVentYSta_enum]  "VHAL_FlashCLEVentYSta_enum"
  Demux1/207 -> Data Type Conversion247/1
  Demux1/213 -> Data Type Conversion240/1
  Demux1/208 -> Data Type Conversion248/1
  Demux1/201 -> Data Type Conversion233/1
  Data Type Conversion246/1 -> [VHAL_FlashCLEVentZSta_enum]  "VHAL_FlashCLEVentZSta_enum"
  Data Type Conversion143/1 -> [VHAL_FlashIVIPTGUSStaSW_enum]  "VHAL_FlashIVIPTGUSStaSW_enum"
  Data Type Conversion139/1 -> [VHAL_FlashLockSetting_enum]  "VHAL_FlashLockSetting_enum"
  Demux1/107 -> Data Type Conversion139/1
  Data Type Conversion141/1 -> [VHAL_FlashRoomLampMode_enum]  "VHAL_FlashRoomLampMode_enum"
  Demux1/109 -> Data Type Conversion141/1
  Data Type Conversion255/1 -> [VHAL_FlashFollowMeENFun_enum]  "VHAL_FlashFollowMeENFun_enum"
  Data Type Conversion253/1 -> [VHAL_FlashWalkInUnLkEN_enum]  "VHAL_FlashWalkInUnLkEN_enum"
  Demux1/222 -> Data Type Conversion255/1
  Demux1/221 -> Data Type Conversion253/1
  Data Type Conversion252/1 -> [VHAL_FlashWalkOutLkEN_enum]  "VHAL_FlashWalkOutLkEN_enum"
  Demux1/220 -> Data Type Conversion252/1
  Bitwise OR15/1 -> Data Type Conversion259/1
  Data Type Conversion256/1 -> Shift Arithmetic43/1
  Data Type Conversion254/1 -> Bitwise OR15/1
  Shift Arithmetic43/1 -> Bitwise OR15/2
  Demux1/223 -> Data Type Conversion254/1
  Demux1/224 -> Data Type Conversion256/1
  Shift Arithmetic44/1 -> Bitwise OR16/2
  Data Type Conversion257/1 -> Bitwise OR16/1
  Data Type Conversion258/1 -> Shift Arithmetic44/1
  Bitwise OR16/1 -> Data Type Conversion260/1
  Demux1/226 -> Data Type Conversion258/1
  Demux1/225 -> Data Type Conversion257/1
  Bitwise OR18/1 -> Data Type Conversion266/1
  Data Type Conversion264/1 -> Shift Arithmetic46/1
  Data Type Conversion263/1 -> Bitwise OR18/1
  Shift Arithmetic46/1 -> Bitwise OR18/2
  Shift Arithmetic45/1 -> Bitwise OR17/2
  Data Type Conversion261/1 -> Bitwise OR17/1
  Data Type Conversion262/1 -> Shift Arithmetic45/1
  Bitwise OR17/1 -> Data Type Conversion265/1
  Bitwise OR19/1 -> Data Type Conversion271/1
  Data Type Conversion268/1 -> Shift Arithmetic47/1
  Data Type Conversion267/1 -> Bitwise OR19/1
  Shift Arithmetic47/1 -> Bitwise OR19/2
  Shift Arithmetic48/1 -> Bitwise OR20/2
  Data Type Conversion269/1 -> Bitwise OR20/1
  Data Type Conversion270/1 -> Shift Arithmetic48/1
  Bitwise OR20/1 -> Data Type Conversion272/1
  Demux1/227 -> Data Type Conversion261/1
  Demux1/228 -> Data Type Conversion262/1
  Demux1/229 -> Data Type Conversion263/1
  Demux1/230 -> Data Type Conversion264/1
  Demux1/231 -> Data Type Conversion267/1
  Demux1/232 -> Data Type Conversion268/1
  Demux1/233 -> Data Type Conversion269/1
  Demux1/234 -> Data Type Conversion270/1
  Data Type Conversion259/1 -> [VHAL_FlashPTGUserHeight1_cnt]  "VHAL_FlashPTGUserHeight1_cnt"
  Data Type Conversion260/1 -> [VHAL_FlashPTGUserHeight2_cnt]  "VHAL_FlashPTGUserHeight2_cnt"
  Data Type Conversion265/1 -> [VHAL_FlashPTGUserHeight3_cnt]  "VHAL_FlashPTGUserHeight3_cnt"
  Data Type Conversion266/1 -> [VHAL_FlashPTGUserHeight4_cnt]  "VHAL_FlashPTGUserHeight4_cnt"
  Data Type Conversion271/1 -> [VHAL_FlashPTGUserHeight5_cnt]  "VHAL_FlashPTGUserHeight5_cnt"
  Data Type Conversion272/1 -> [VHAL_FlashPTGUserHeight7_cnt]  "VHAL_FlashPTGUserHeight7_cnt"
  Demux1/235 -> Data Type Conversion273/1
  Demux1/237 -> Data Type Conversion275/1
  Demux1/236 -> Data Type Conversion274/1
  Data Type Conversion273/1 -> [VHAL_FlashPTGOpenHeight12_enum]  "VHAL_FlashPTGOpenHeight12_enum"
  Data Type Conversion274/1 -> [VHAL_FlashPTGOpenHeight34_enum]  "VHAL_FlashPTGOpenHeight34_enum"
  Data Type Conversion275/1 -> [VHAL_FlashPTGOpenHeight57_enum]  "VHAL_FlashPTGOpenHeight57_enum"
  u8_TPMSSensorIDRegSta/1 -> [VHAL_TPMSSensorIDRegSta_raw]  "VHAL_TPMSSensorIDRegSta_raw"
  Data Type Conversion280/1 -> [VHAL_DIDFlashAutoWipHSpdEN_raw8]
  Data Type Conversion282/1 -> [VHAL_DIDFlashWipRLSCmdCutFilter_raw8]
  Demux1/243 -> Data Type Conversion282/1
  Demux1/241 -> Data Type Conversion280/1
  Demux1/245 -> Data Type Conversion291/1
  Data Type Conversion291/1 -> [VHAL_FlashAutoUnlock_enum]  "VHAL_FlashAutoUnlock_enum"
  Demux1/244 -> Data Type Conversion290/1
  Data Type Conversion290/1 -> [VHAL_FlashAutoLock_enum]  "VHAL_FlashAutoLock_enum"
  Demux1/242 -> Data Type Conversion281/1
  Data Type Conversion281/1 -> [VHAL_DIDFlashWipRLSCmdHoldFilter_raw8]
  Demux1/238 -> Data Type Conversion276/1
  Demux1/239 -> Data Type Conversion277/1
  Demux1/240 -> Data Type Conversion278/1
  Data Type Conversion276/1 -> [VHAL_FlashACCLevelSta12_enum]  "VHAL_FlashACCLevelSta12_enum"
  Data Type Conversion277/1 -> [VHAL_FlashACCLevelSta34_enum]  "VHAL_FlashACCLevelSta34_enum"
  Data Type Conversion278/1 -> [VHAL_FlashACCLevelSta57_enum]  "VHAL_FlashACCLevelSta57_enum"
  [VHAL_DIDFlashDKCKey_raw8] -> DIDGet_List/3(VHAL_DIDFlashDKCKey_raw8)
  [VHAL_DIDFlashAutoWipHSpdEN_raw8] -> DIDGet_List/12(VHAL_DIDFlashAutoWipHSpdEN_raw8)
  Bus Selector/7 -> [VHAL_DIDGetTurnLampRLThreCurr_raw8]  "<VHAL_DIDGetTurnLampRLThreCurr_raw8>"
  [VHAL_DIDFlashWipRLSCmdHoldFilter_raw8] -> DIDGet_List/13(VHAL_DIDFlashWipRLSCmdHoldFilter_raw8)
  Bus Selector/1 -> [VHAL_DIDGetXWDMode_raw8]  "<VHAL_DIDGetXWDMode_raw8>"
  [VHAL_DIDFlashWipRLSCmdCutFilter_raw8] -> DIDGet_List/14(VHAL_DIDFlashWipRLSCmdCutFilter_raw8)
  [VHAL_DIDFlashUSSConfig_raw8] -> DIDGet_List/15(VHAL_DIDFlashUSSConfig_raw8)
  [VHAL_DIDFlashTireSize_raw8] -> DIDGet_List/16(VHAL_DIDFlashTireSize_raw8)
  Bus Selector/13 -> [VHAL_DIDGetWipRLSCmdCutFilter_raw8]  "<VHAL_DIDGetWipRLSCmdCutFilter_raw8>"
  Ground1/1 -> DIDGet_List/4(VHAL_DIDFlashDynoMode_raw8)
  Bus Selector/12 -> [VHAL_DIDGetWipRLSCmdHoldFilter_raw8]  "<VHAL_DIDGetWipRLSCmdHoldFilter_raw8>"
  [VHAL_DIDFlashXWDMode_raw8] -> DIDGet_List/2(VHAL_DIDFlashXWDMode_raw8)
  Bus Selector/6 -> [VHAL_DIDGetTurnLampFLThreCurr_raw8]  "<VHAL_DIDGetTurnLampFLThreCurr_raw8>"
  Bus Selector/15 -> [VHAL_DIDGetTireSize_raw8]  "<VHAL_DIDGetTireSize_raw8>"
  [VHAL_DIDFlashTurnLampRRThreCurr_raw8] -> DIDGet_List/6(VHAL_DIDFlashTurnLampRRThreCurr_raw8)
  Bus Selector/2 -> [VHAL_DIDGetDKCKey_raw8]  "<VHAL_DIDGetDKCKey_raw8>"
  [VHAL_DIDFlashTurnLampFRThreCurr_raw8] -> DIDGet_List/5(VHAL_DIDFlashTurnLampFRThreCurr_raw8)
  Bus Selector/11 -> [VHAL_DIDGetAutoWipHSpdEN_raw8]  "<VHAL_DIDGetAutoWipHSpdEN_raw8>"
  [VHAL_DIDFlashTurnLampRLThreCurr_raw8] -> DIDGet_List/8(VHAL_DIDFlashTurnLampRLThreCurr_raw8)
  [VHAL_DIDFlashDRLDis_raw8] -> DIDGet_List/11(VHAL_DIDFlashDRLDis_raw8)
  [VHAL_DIDFlashTurnLampFLThreCurr_raw8] -> DIDGet_List/7(VHAL_DIDFlashTurnLampFLThreCurr_raw8)
  Bus Selector/16 -> [VHAL_DIDGetAPSFunConfig_raw8]  "<VHAL_DIDGetAPSFunConfig_raw8>"
  Bus Selector/9 -> [VHAL_DIDGetAutoLock_raw8]  "<VHAL_DIDGetAutoLock_raw8>"
  [VHAL_DIDFlashFMHTimer_raw8] -> DIDGet_List/9(VHAL_DIDFlashFMHTimer_raw8)
  Bus Selector/10 -> [VHAL_DIDGetDRLDis_raw8]  "<VHAL_DIDGetDRLDis_raw8>"
  DIDGet_List/1(BHAL_DIDOrigOutput_raw8) -> [BHAL_DIDOrigOutput_raw8]
  [VHAL_DIDFlashAutoLock_raw8] -> DIDGet_List/10(VHAL_DIDFlashAutoLock_raw8)
  [VHAL_DIDFlashAPSFunConfig_raw8] -> DIDGet_List/17(VHAL_DIDFlashAPSFunConfig_raw8)
  Bus Selector/4 -> [VHAL_DIDGetTurnLampFRThreCurr_raw8]  "<VHAL_DIDGetTurnLampFRThreCurr_raw8>"
  Bus Selector/5 -> [VHAL_DIDGetTurnLampRRThreCurr_raw8]  "<VHAL_DIDGetTurnLampRRThreCurr_raw8>"
  Bus Selector/14 -> [VHAL_DIDGetUSSConfig_raw8]  "<VHAL_DIDGetUSSConfig_raw8>"
  Bus Selector/8 -> [VHAL_DIDGetFMHTimer_raw8]  "<VHAL_DIDGetFMHTimer_raw8>"
  [BHAL_DIDOrigOutput_raw8] -> Bus Selector/1
  [BHAL_DIDGetData_raw] -> DIDGet_List/1(BHAL_DIDGetData_raw)
  Bus Selector/3 -> [VHAL_DIDGetDynoMode_raw8]  "<VHAL_DIDGetDynoMode_raw8>"
  VHAL_ResetPedalZeroPosReq_raw/1 -> [VHAL_ResetPedalZeroPosReq_raw]
  [VHAL_ResetPedalZeroPosReq_raw] -> Data Type Conversion279/1
  Data Type Conversion165/1 -> Bus Creator/75  "VHAL_Pedal1Ref5V_V"
  Data Type Conversion166/1 -> Bus Creator/76  "VHAL_Pedal2Ref5V_V"
  Data Type Conversion31/1 -> Bus Creator/71  "VHAL_AnyNMID_flg"
  Data Type Conversion33/1 -> Bus Creator/72  "VHAL_CurrentNmState_enum"
  Data Type Conversion56/1 -> Bus Creator/73  "VHAL_NvmProtectSta_flg"
  Data Type Conversion167/1 -> Bus Creator/74  "VHAL_AuxBattVolmV_mV"
  Data Type Conversion184/1 -> Bus Creator/83  "VHAL_NetworkReqCalled_flg"
  Data Type Conversion187/1 -> Bus Creator/84  "VHAL_PmicBootReason_enum"
  Data Type Conversion186/1 -> Bus Creator/85  "VHAL_WisrBootReason_raw32"
  Data Type Conversion57/1 -> Bus Creator/89  "VHAL_CAN1BusOff_flg"
  Data Type Conversion110/1 -> Bus Creator/90  "VHAL_CAN2BusOff_flg"
  Data Type Conversion188/1 -> Bus Creator/91  "VHAL_CAN3BusOff_flg"
  Data Type Conversion111/1 -> Bus Creator/92  "VHAL_CAN4BusOff_flg"
  Data Type Conversion189/1 -> Bus Creator/93  "VHAL_CAN5BusOff_flg"
  Data Type Conversion292/1 -> Bus Creator/15  "VHAL_ECUGen1_cnt"
  Data Type Conversion293/1 -> Bus Creator/16  "VHAL_ECUGen2_cnt"
  Data Type Conversion17/1 -> Bus Creator/21  "VHAL_Dash1_cnt"
  Data Type Conversion18/1 -> Bus Creator/22  "VHAL_Change1_cnt"
  Data Type Conversion19/1 -> Bus Creator/23  "VHAL_Change2_cnt"
  Data Type Conversion20/1 -> Bus Creator/24  "VHAL_Dash2_cnt"
  Data Type Conversion21/1 -> Bus Creator/25  "VHAL_SHA1_cnt"
  Data Type Conversion22/1 -> Bus Creator/26  "VHAL_SHA2_cnt"
  Data Type Conversion23/1 -> Bus Creator/27  "VHAL_SHA3_cnt"
  Data Type Conversion24/1 -> Bus Creator/28  "VHAL_SHA4_cnt"
  Data Type Conversion25/1 -> Bus Creator/29  "VHAL_SHA5_cnt"
  Data Type Conversion26/1 -> Bus Creator/30  "VHAL_SHA6_cnt"
  Data Type Conversion27/1 -> Bus Creator/31  "VHAL_SHA7_cnt"
  Data Type Conversion28/1 -> Bus Creator/32  "VHAL_SHA8_cnt"
  Data Type Conversion1/1 -> Bus Creator/33  "VHAL_AcoreReadyToSlp_flg"
  Data Type Conversion29/1 -> Bus Creator/34  "VHAL_PwrReq_OTA_enum"
  Data Type Conversion30/1 -> Bus Creator/35  "VHAL_AllowMovThd_OTA_enum"
  Data Type Conversion32/1 -> Bus Creator/36  "VHAL_EvccAplusPwrUpReq_flg"
  [VHAL_FlashHoodSW_flg] -> Bus Creator/79
  [VHAL_FlashTailgateSW_flg] -> Bus Creator/80
  [VHAL_FlashCTDLockSW_flg] -> Bus Creator/81
  [VHAL_FlashTailgateHDSW_flg] -> Bus Creator/82
  [VHAL_FlashAPMDoorControlSta_flg] -> Bus Creator/86
  [VHAL_EAPS1MINMem_pct] -> Bus Creator/77
  [VHAL_EAPS2MINMem_pct] -> Bus Creator/78
  [VHAL_DrivetrainSelect_enum] -> Bus Creator/37
  [VHAL_ReadFlashCorrect_flg] -> Bus Creator/38
  [VHAL_FlashAntitheft_enum] -> Bus Creator/39
  [VHAL_RandomnumberY_raw1] -> Bus Creator/40
  [VHAL_RandomnumberY_raw2] -> Bus Creator/41
  [VHAL_RandomnumberY_raw3] -> Bus Creator/42
  [VHAL_RandomnumberY_raw4] -> Bus Creator/43
  [VHAL_RandomnumberY_raw5] -> Bus Creator/44
  [VHAL_RandomnumberY_raw6] -> Bus Creator/45
  [VHAL_RandomnumberY_raw7] -> Bus Creator/46
  [VHAL_RandomnumberY_raw8] -> Bus Creator/47
  [VHAL_FlashACModeSet123_enum] -> Bus Creator/48
  [VHAL_FlashFace_enum] -> Bus Creator/49
  [VHAL_FlashFoot_enum] -> Bus Creator/50
  [VHAL_FlashFrost_enum] -> Bus Creator/51
  [VHAL_FlashFaceM_enum] -> Bus Creator/52
  [VHAL_FlashFootM_enum] -> Bus Creator/53
  [VHAL_FlashCCUSyncSts_enum] -> Bus Creator/54
  [VHAL_FlashACForceOFF_flg] -> Bus Creator/55
  [VHAL_FlashsigRecircSt_enum] -> Bus Creator/56
  [VHAL_FlashRecAutoFlg_enum] -> Bus Creator/57
  [VHAL_FlashAirIntenZone1M_enum] -> Bus Creator/58
  [VHAL_Flashfdefog_enum] -> Bus Creator/59
  [VHAL_FlashsigSetTempZon1St_C] -> Bus Creator/60
  [VHAL_FlashsigSetTempZon2StM_C] -> Bus Creator/61
  [VHAL_FlashCountAlarm_enum] -> Bus Creator/62
  [VHAL_FlashMFSWTri_flg] -> Bus Creator/63
  [VHAL_FlashMirrorFlodPos_flg] -> Bus Creator/64
  [VHAL_FlashFuelDoorPos_flg] -> Bus Creator/65
  [VHAL_FlashLockSetting_enum] -> Bus Creator/66
  [VHAL_FlashMFRDNBrightReq_pct] -> Bus Creator/67
  [VHAL_FlashRoomLampMode_enum] -> Bus Creator/68
  [VHAL_FlashWiperFixMode_flg] -> Bus Creator/69
  [VHAL_FlashIVIPTGUSStaSW_enum] -> Bus Creator/70
  [VHAL_AcoreRebootCmd_flg] -> Bus Creator/87  "VHAL_AcoreRebootCmd_flg"
  [VHAL_DIDGetDynoMode_flg] -> Bus Creator/88
  Demux/15 -> Data Type Conversion292/1
  Demux/16 -> Data Type Conversion293/1
  Switch13/1 -> Data Type Conversion285/1
  Logical Operator10/1 -> Switch12/2
  Logical Operator11/1 -> Switch13/2
  Data Type Conversion286/1 -> Equal37/1, Equal36/1, Bit Shift/1, Switch14/3
  Bit Shift/1 -> Bitwise AND1/1
  Data Type Conversion288/1 -> [VHAL_WipRLSCmdCutTime_s]  "VHAL_WipRLSCmdCutTime_s"
  Constant44/1 -> Equal32/2
  Bitwise AND3/1 -> Equal32/1, Equal33/1, Switch12/3
  Bitwise AND2/1 -> Data Type Conversion287/1
  Switch15/1 -> Bitwise AND2/1
  Constant47/1 -> Equal35/2
  Data Type Conversion289/1 -> Bit Shift1/1, Switch15/3, Equal39/1, Equal38/1
  Data Type Conversion287/1 -> [VHAL_WipRLSCmdCutEN_flg]  "VHAL_WipRLSCmdCutEN_flg"
  [VHAL_DIDGetWipRLSCmdCutFilter_raw8] -> Data Type Conversion289/1
  Switch12/1 -> Data Type Conversion288/1
  Constant54/1 -> Equal38/2
  Logical Operator12/1 -> Switch14/2
  Constant46/1 -> Switch12/1
  Constant53/1 -> Equal39/2
  Constant48/1 -> Equal34/2
  Constant52/1 -> Switch14/1
  Bitwise AND1/1 -> Switch13/3, Equal35/1, Equal34/1
  Data Type Conversion285/1 -> [VHAL_WipRLSCmdHoldTime_s]  "VHAL_WipRLSCmdHoldTime_s"
  Constant43/1 -> Equal33/2
  Equal39/1 -> Logical Operator13/2
  Equal33/1 -> Logical Operator10/2
  Equal38/1 -> Logical Operator13/1
  Switch14/1 -> Bitwise AND/1
  Constant49/1 -> Switch13/1
  Constant55/1 -> Switch15/1
  Equal36/1 -> Logical Operator12/1
  Equal37/1 -> Logical Operator12/2
  Logical Operator13/1 -> Switch15/2
  Constant51/1 -> Equal36/2
  [VHAL_DIDGetWipRLSCmdHoldFilter_raw8] -> Data Type Conversion286/1
  Constant50/1 -> Equal37/2
  Data Type Conversion284/1 -> [VHAL_WipRLSCmdHoldEN_flg]  "VHAL_WipRLSCmdHoldEN_flg"
  Bit Shift1/1 -> Bitwise AND3/1
  Bitwise AND/1 -> Data Type Conversion284/1
  Equal35/1 -> Logical Operator11/2
  Equal32/1 -> Logical Operator10/1
  Equal34/1 -> Logical Operator11/1
  Constant41/1 -> Equal26/2
  [VHAL_DIDGetAutoWipHSpdEN_raw8] -> Equal26/1
  Constant33/1 -> Equal27/2
  Switch11/1 -> Data Type Conversion283/1
  Equal26/1 -> Logical Operator9/1
  Equal27/1 -> Logical Operator9/2
  Data Type Conversion283/1 -> [VHAL_AutoWipHSpdEN_flg]  "VHAL_AutoWipHSpdEN_flg"
  [VHAL_DIDGetAutoWipHSpdEN_raw8] -> Equal27/1
  Logical Operator9/1 -> Switch11/2
  Constant42/1 -> Switch11/1
  [VHAL_DIDGetAutoWipHSpdEN_raw8] -> Switch11/3
  [VHAL_VinCode_raw] -> Data Type Conversion814/1
  Data Type Conversion294/1 -> Bus Creator/94  "VHAL_CAN6BusOff_flg"
  [VHAL_CAN6BusOff_flg] -> Data Type Conversion294/1
  Data Type Conversion814/1 -> Bus Creator/234  "VHAL_VinCode_cnt"
  Data Type Conversion213/1 -> Bus Creator/106  "VHAL_FlashRegenMode_enum"
  Data Type Conversion279/1 -> Bus Creator/148  "VHAL_ResetPedalZeroPosReq_enum"
  [VHAL_FlashPTGOpenHeight12_enum] -> Bus Creator/155
  [VHAL_FlashPTGOpenHeight34_enum] -> Bus Creator/156
  [VHAL_FlashPTGOpenHeight57_enum] -> Bus Creator/157
  [VHAL_FlashACCLevelSta12_enum] -> Bus Creator/158
  [VHAL_FlashACCLevelSta34_enum] -> Bus Creator/159
  [VHAL_FlashACCLevelSta57_enum] -> Bus Creator/160
  [VHAL_AutoWipHSpdEN_flg] -> Bus Creator/161
  [VHAL_WipRLSCmdHoldEN_flg] -> Bus Creator/162
  [VHAL_WipRLSCmdHoldTime_s] -> Bus Creator/163
  [VHAL_WipRLSCmdCutEN_flg] -> Bus Creator/164
  [VHAL_WipRLSCmdCutTime_s] -> Bus Creator/165
  [VHAL_FlashAutoLock_enum] -> Bus Creator/166
  [VHAL_FlashAutoUnlock_enum] -> Bus Creator/167
  [VHAL_PmicBootPath_raw32] -> Bus Creator/168
  [VHAL_FlashTPMModelVersion_raw] -> Bus Creator/169
  [VHAL_FlashTPMModelVersionChkSum_raw] -> Bus Creator/170
  [VHAL_FlashMILDIST_km] -> Bus Creator/171  "VHAL_FlashMILDIST_km"
  [VHAL_FlashWARMUPS_cnt] -> Bus Creator/172  "VHAL_FlashWARMUPS_cnt"
  [VHAL_FlashCLRDIST_km] -> Bus Creator/173  "VHAL_FlashCLRDIST_km"
  [VHAL_FlashMILTIME_min] -> Bus Creator/174  "VHAL_FlashMILTIME_min"
  [VHAL_FlashCLRTIME_min] -> Bus Creator/175  "VHAL_FlashCLRTIME_min"
  [VHAL_FlashNUMPSATRIPSFLTMEMCLR_cnt] -> Bus Creator/176  "VHAL_FlashNUMPSATRIPSFLTMEMCLR_cnt"
  [VHAL_FlashODOMETER_km] -> Bus Creator/177  "VHAL_FlashODOMETER_km"
  [VHAL_FlashPSAR_sec] -> Bus Creator/178  "VHAL_FlashPSAR_sec"
  [VHAL_FlashPSAL_sec] -> Bus Creator/179  "VHAL_FlashPSAL_sec"
  [VHAL_FlashIPSAR_sec] -> Bus Creator/180  "VHAL_FlashIPSAR_sec"
  [VHAL_FlashIPSAL_sec] -> Bus Creator/181  "VHAL_FlashIPSAL_sec"
  [VHAL_FlashCPSAR_sec] -> Bus Creator/182  "VHAL_FlashCPSAR_sec"
  [VHAL_FlashCPSAL_sec] -> Bus Creator/183  "VHAL_FlashCPSAL_sec"
  [VHAL_FlashHVBNAH_Ahr] -> Bus Creator/184  "VHAL_FlashHVBNAH_Ahr"
  [VHAL_FlashHVBNE_kWh] -> Bus Creator/185  "VHAL_FlashHVBNE_kWh"
  [VHAL_FlashIGNCNTR_cnt] -> Bus Creator/186  "VHAL_FlashIGNCNTR_cnt"
  [VHAL_FlashTNBCPSAR_Ahr] -> Bus Creator/187  "VHAL_FlashTNBCPSAR_Ahr"
  [VHAL_FlashTNBCPSAL_Ahr] -> Bus Creator/188  "VHAL_FlashTNBCPSAL_Ahr"
  [VHAL_FlashTNECPSAR_kWh] -> Bus Creator/189  "VHAL_FlashTNECPSAR_kWh"
  [VHAL_FlashTNECPSAL_kWh] -> Bus Creator/190  "VHAL_FlashTNECPSAL_kWh"
  [VHAL_FlashTEBPSAR_kWh] -> Bus Creator/191  "VHAL_FlashTEBPSAR_kWh"
  [VHAL_FlashTEBPSAL_kWh] -> Bus Creator/192  "VHAL_FlashTEBPSAL_kWh"
  [VHAL_FlashTGEOVCR_kWh] -> Bus Creator/193  "VHAL_FlashTGEOVCR_kWh"
  [VHAL_FlashTGEOVCL_kWh] -> Bus Creator/194  "VHAL_FlashTGEOVCL_kWh"
  [VHAL_FlashGECHGOVCDCR_kWh] -> Bus Creator/195  "VHAL_FlashGECHGOVCDCR_kWh"
  [VHAL_FlashGECHGOVCDCL_kWh] -> Bus Creator/196  "VHAL_FlashGECHGOVCDCL_kWh"
  [VHAL_FlashGECHGOVCACR_kWh] -> Bus Creator/197  "VHAL_FlashGECHGOVCACR_kWh"
  [VHAL_FlashGECHGOVCACL_kWh] -> Bus Creator/198  "VHAL_FlashGECHGOVCACL_kWh"
  [VHAL_FlashRESSV2XENNONPSAR_kWh] -> Bus Creator/199  "VHAL_FlashRESSV2XENNONPSAR_kWh"
  [VHAL_FlashRESSV2XENNONPSAL_kWh] -> Bus Creator/200  "VHAL_FlashRESSV2XENNONPSAL_kWh"
  [VHAL_FlashPKERNumerator_kphsqr] -> Bus Creator/201  "VHAL_FlashPKERNumerator_kphsqr"
  [VHAL_FlashPKELNumerator_kphsqr] -> Bus Creator/202  "VHAL_FlashPKELNumerator_kphsqr"
  [VHAL_FlashResetCDEODTR_km] -> Bus Creator/203  "VHAL_FlashResetCDEODTR_km"
  [VHAL_FlashAvgBattTempPSAR_C] -> Bus Creator/204  "VHAL_FlashAvgBattTempPSAR_C"
  [VHAL_FlashAvgBattTempPSAL_C] -> Bus Creator/205  "VHAL_FlashAvgBattTempPSAL_C"
  [VHAL_FlashAvgBattTempOVCR_C] -> Bus Creator/206  "VHAL_FlashAvgBattTempOVCR_C"
  [VHAL_FlashAvgBattTempOVCL_C] -> Bus Creator/207  "VHAL_FlashAvgBattTempOVCL_C"
  [VHAL_FlashAvgBattTempOFFR_C] -> Bus Creator/208  "VHAL_FlashAvgBattTempOFFR_C"
  [VHAL_FlashAvgBattTempOFFL_C] -> Bus Creator/209  "VHAL_FlashAvgBattTempOFFL_C"
  [VHAL_FlashQTYPSATRIPSR_cnt] -> Bus Creator/210  "VHAL_FlashQTYPSATRIPSR_cnt"
  [VHAL_FlashQTYPSATRIPSL_cnt] -> Bus Creator/211  "VHAL_FlashQTYPSATRIPSL_cnt"
  [VHAL_FlashRESSCNTDODRNGR_cnt] -> Bus Creator/212  "VHAL_FlashRESSCNTDODRNGR_cnt"
  [VHAL_FlashRESSCNTDODRNGL_cnt] -> Bus Creator/213  "VHAL_FlashRESSCNTDODRNGL_cnt"
  [VHAL_FlashETMATOER_kWh] -> Bus Creator/214  "VHAL_FlashETMATOER_kWh"
  [VHAL_FlashETMATOEL_kWh] -> Bus Creator/215  "VHAL_FlashETMATOEL_kWh"
  [VHAL_FlashETMBTOER_kWh] -> Bus Creator/216  "VHAL_FlashETMBTOER_kWh"
  [VHAL_FlashETMBTOEL_kWh] -> Bus Creator/217  "VHAL_FlashETMBTOEL_kWh"
  [VHAL_FlashRESSTIMESOCPSARNGR_s] -> Bus Creator/218  "VHAL_FlashRESSTIMESOCPSARNGR_s"
  [VHAL_FlashRESSTIMESOCPSARNGL_s] -> Bus Creator/219  "VHAL_FlashRESSTIMESOCPSARNGL_s"
  [VHAL_FlashRESSTIMESOCCHGRNGR_s] -> Bus Creator/220  "VHAL_FlashRESSTIMESOCCHGRNGR_s"
  [VHAL_FlashRESSTIMESOCCHGRNGL_s] -> Bus Creator/221  "VHAL_FlashRESSTIMESOCCHGRNGL_s"
  [VHAL_FlashRESSTIMESOCOFFRNGR_s] -> Bus Creator/222  "VHAL_FlashRESSTIMESOCOFFRNGR_s"
  [VHAL_FlashRESSTIMESOCOFFRNGL_s] -> Bus Creator/223  "VHAL_FlashRESSTIMESOCOFFRNGL_s"
  [VHAL_FlashMAXBATTEMPL_C] -> Bus Creator/224  "VHAL_FlashMAXBATTEMPL_C"
  [VHAL_FlashMINBATTEMPL_C] -> Bus Creator/225  "VHAL_FlashMINBATTEMPL_C"
  [VHAL_FlashAVGBATTEMPL_sec] -> Bus Creator/226  "VHAL_FlashAVGBATTEMPL_sec"
  [VHAL_FlashAVGBATTEMPL_C] -> Bus Creator/227  "VHAL_FlashAVGBATTEMPL_C"
  [VHAL_FlashBattTempPSAR_sec] -> Bus Creator/228  "VHAL_FlashBattTempPSAR_sec"
  [VHAL_FlashBattTempPSAL_sec] -> Bus Creator/229  "VHAL_FlashBattTempPSAL_sec"
  [VHAL_FlashOVCR_sec] -> Bus Creator/230  "VHAL_FlashOVCR_sec"
  [VHAL_FlashOVCL_sec] -> Bus Creator/231  "VHAL_FlashOVCL_sec"
  [VHAL_FlashOFFR_sec] -> Bus Creator/232  "VHAL_FlashOFFR_sec"
  [VHAL_FlashOFFL_sec] -> Bus Creator/233  "VHAL_FlashOFFL_sec"
  [VHAL_FlashAmbFunEN_enum] -> Bus Creator/107
  [VHAL_FlashAmbWelEN_enum] -> Bus Creator/108
  [VHAL_FlashAmbDimEN_enum] -> Bus Creator/109
  [VHAL_FlashAmbLinkDriSta_enum] -> Bus Creator/110
  [VHAL_FlashAmbPwrWarnEN_enum] -> Bus Creator/111
  [VHAL_FlashAmbODAEN_enum] -> Bus Creator/112
  [VHAL_FlashAmbColorSta1_enum] -> Bus Creator/113
  [VHAL_FlashAmbColorSta2_enum] -> Bus Creator/114
  [VHAL_FlashAmbColorSta3_enum] -> Bus Creator/115
  [VHAL_FlashAmbColorSta4_enum] -> Bus Creator/116
  [VHAL_FlashAmbColorSta5_enum] -> Bus Creator/117
  [VHAL_FlashAmbColorSta7_enum] -> Bus Creator/118
  [VHAL_FlashAmbBrightnessSta1_enum] -> Bus Creator/119
  [VHAL_FlashAmbBrightnessSta2_enum] -> Bus Creator/120
  [VHAL_FlashAmbBrightnessSta3_enum] -> Bus Creator/121
  [VHAL_FlashAmbBrightnessSta4_enum] -> Bus Creator/122
  [VHAL_FlashAmbBrightnessSta5_enum] -> Bus Creator/123
  [VHAL_FlashAmbBrightnessSta7_enum] -> Bus Creator/124
  [VHAL_FlashTurnSwTSet123_enum] -> Bus Creator/125
  [VHAL_FlashTurnSwTSet457_enum] -> Bus Creator/126
  [VHAL_FlashAirIntZ3Sta_enum] -> Bus Creator/127
  [VHAL_FlashPsEVentModeSta_enum] -> Bus Creator/128
  [VHAL_FlashDrEVentModeSta_enum] -> Bus Creator/129
  [VHAL_FlashDrEVentZSta_enum] -> Bus Creator/130
  [VHAL_FlashCLEVentZSta_enum] -> Bus Creator/131
  [VHAL_FlashPsEVentZSta_enum] -> Bus Creator/132
  [VHAL_FlashCREVentZSta_enum] -> Bus Creator/133
  [VHAL_FlashDrVentEN_enum] -> Bus Creator/134
  [VHAL_FlashDrEVentYSta_enum] -> Bus Creator/135
  [VHAL_FlashCLVentEN_enum] -> Bus Creator/136
  [VHAL_FlashCLEVentYSta_enum] -> Bus Creator/137
  [VHAL_FlashPsVentEN_enum] -> Bus Creator/138
  [VHAL_FlashPsEVentYSta_enum] -> Bus Creator/139
  [VHAL_FlashCRVentEN_enum] -> Bus Creator/140
  [VHAL_FlashCREVentYSta_enum] -> Bus Creator/141
  [VHAL_FlashFGSAirIntSta_enum] -> Bus Creator/142
  [VHAL_FlashFGSChSta_enum] -> Bus Creator/143
  [VHAL_FlashFGSIONSWSta_enum] -> Bus Creator/144
  [VHAL_FlashWalkOutLkEN_enum] -> Bus Creator/145
  [VHAL_FlashWalkInUnLkEN_enum] -> Bus Creator/146
  [VHAL_FlashFollowMeENFun_enum] -> Bus Creator/147
  [VHAL_FlashPTGUserHeight1_cnt] -> Bus Creator/149
  [VHAL_FlashPTGUserHeight2_cnt] -> Bus Creator/150
  [VHAL_FlashPTGUserHeight3_cnt] -> Bus Creator/151
  [VHAL_FlashPTGUserHeight4_cnt] -> Bus Creator/152
  [VHAL_FlashPTGUserHeight5_cnt] -> Bus Creator/153
  [VHAL_FlashPTGUserHeight7_cnt] -> Bus Creator/154
  [VHAL_funAuto_flg] -> Bus Creator/95
  [VHAL_DiagDRLOFF_flg] -> Bus Creator/96
  [VHAL_DiagFMHT_s] -> Bus Creator/97
  [VHAL_DiagFLTC_mA] -> Bus Creator/98
  [VHAL_DiagFRTC_mA] -> Bus Creator/99
  [VHAL_DiagRLTC_mA] -> Bus Creator/100
  [VHAL_DiagRRTC_mA] -> Bus Creator/101
  [VHAL_USSConfig_raw8] -> Bus Creator/102  "VHAL_USSConfig_raw8"
  [VHAL_TireSize_raw8] -> Bus Creator/103  "VHAL_TireSize_raw8"
  [VHAL_APSFunConfig_raw8] -> Bus Creator/104  "VHAL_APSFunConfig_raw8"
  [VHAL_FlashfUnlockSingle_flg] -> Bus Creator/105
  VHAL_CAN6BusOff_raw/1 -> [VHAL_CAN6BusOff_raw]
  VHAL_PmicBootPath_raw32/1 -> Data Type Conversion295/1
  Data Type Conversion295/1 -> [VHAL_PmicBootPath_raw32]  "VHAL_PmicBootPath_raw32"
  Constant56/1 -> LatchedFlg/2
  LatchedFlg3/1 -> [VHAL_CAN4BusOff_flg]
  [VHAL_CAN6BusOff_raw] -> LatchedFlg5/1
  LatchedFlg2/1 -> [VHAL_CAN3BusOff_flg]
  [VHAL_CAN3BusOff_raw] -> LatchedFlg2/1
  LatchedFlg1/1 -> [VHAL_CAN2BusOff_flg]
  Constant62/1 -> LatchedFlg3/2
  [VHAL_CAN4BusOff_raw] -> LatchedFlg3/1
  Constant64/1 -> LatchedFlg4/2
  LatchedFlg5/1 -> [VHAL_CAN6BusOff_flg]
  [VHAL_CAN1BusOff_raw] -> LatchedFlg/1
  Constant57/1 -> LatchedFlg/3
  Constant65/1 -> LatchedFlg4/3
  Constant59/1 -> LatchedFlg1/3
  Constant66/1 -> LatchedFlg5/2
  Constant58/1 -> LatchedFlg1/2
  Constant61/1 -> LatchedFlg2/3
  [VHAL_CAN2BusOff_raw] -> LatchedFlg1/1
  LatchedFlg/1 -> [VHAL_CAN1BusOff_flg]
  Constant63/1 -> LatchedFlg3/3
  [VHAL_CAN5BusOff_raw] -> LatchedFlg4/1
  Constant67/1 -> LatchedFlg5/3
  Constant60/1 -> LatchedFlg2/2
  LatchedFlg4/1 -> [VHAL_CAN5BusOff_flg]
  Data Type Conversion297/1 -> [VHAL_FlashTPMModelVersionChkSum_raw]  "VHAL_FlashTPMModelVersionChkSum_raw"
  Data Type Conversion296/1 -> [VHAL_FlashTPMModelVersion_raw]  "VHAL_FlashTPMModelVersion_raw"
  Demux1/246 -> Data Type Conversion296/1
  Demux1/247 -> Data Type Conversion297/1
  Demux1/250 -> Data Type Conversion817/1
  Data Type Conversion819/1 -> [VHAL_FlashHMIKey5Func_enum]  "VHAL_FlashHMIKey5Func_enum"
  Demux1/249 -> Data Type Conversion816/1
  Demux1/253 -> Data Type Conversion820/1
  Demux1/248 -> Data Type Conversion815/1
  Demux1/254 -> Data Type Conversion821/1
  Demux1/252 -> Data Type Conversion819/1
  Data Type Conversion823/1 -> [VHAL_FlashAutoWipHSpdEN_flg]  "VHAL_FlashAutoWipHSpdEN_flg"
  Data Type Conversion816/1 -> [VHAL_FlashHMIKey2Func_enum]  "VHAL_FlashHMIKey2Func_enum"
  Data Type Conversion817/1 -> [VHAL_FlashHMIKey3Func_enum]  "VHAL_FlashHMIKey3Func_enum"
  Demux1/251 -> Data Type Conversion818/1
  Data Type Conversion820/1 -> [VHAL_FlashHMIKey6Func_enum]  "VHAL_FlashHMIKey6Func_enum"
  Data Type Conversion818/1 -> [VHAL_FlashHMIKey4Func_enum]  "VHAL_FlashHMIKey4Func_enum"
  Demux1/255 -> Data Type Conversion822/1
  Demux1/256 -> Data Type Conversion823/1
  Data Type Conversion821/1 -> [VHAL_FlashHMIKey7Func_enum]  "VHAL_FlashHMIKey7Func_enum"
  Data Type Conversion822/1 -> [VHAL_FlashHMIKey8Func_enum]  "VHAL_FlashHMIKey8Func_enum"
  Data Type Conversion815/1 -> [VHAL_FlashHMIKey1Func_enum]  "VHAL_FlashHMIKey1Func_enum"
  Data Type Conversion298/1 -> [VHAL_DIDGetDynoMode_flg]  "VHAL_DIDGetDynoMode_flg"
  [VHAL_TPMSSensorIDRegSta_raw] -> Bus Creator/277
  [VHAL_FlashIDvaild_enum] -> Bus Creator/276
  [VHAL_FlashS4ID_raw] -> Bus Creator/275
  [VHAL_FlashS3ID_raw] -> Bus Creator/274
  [VHAL_FlashS2ID_raw] -> Bus Creator/273
  [VHAL_FlashS1ID_raw] -> Bus Creator/272
  [VHAL_Prepresstempvalid_enum] -> Bus Creator/271
  [VHAL_unlearnSfailvalid_enum] -> Bus Creator/270
  [VHAL_unlearnSfali_flg] -> Bus Creator/269
  [VHAL_RRWheelTemp_C] -> Bus Creator/268
  [VHAL_LRWheelTemp_C] -> Bus Creator/267
  [VHAL_RFWheelTemp_C] -> Bus Creator/266
  [VHAL_LFWheelTemp_C] -> Bus Creator/265
  [VHAL_RRWheelPress_raw8] -> Bus Creator/264
  [VHAL_LRWheelPress_raw8] -> Bus Creator/263
  [VHAL_RFWheelPress_raw8] -> Bus Creator/262
  [VHAL_LFWheelPress_raw8] -> Bus Creator/261
  [VHAL_RRP20_raw8] -> Bus Creator/260
  [VHAL_LRP20_raw8] -> Bus Creator/259
  [VHAL_RFP20_raw8] -> Bus Creator/258
  [VHAL_LFP20_raw8] -> Bus Creator/257
  [VHAL_RRPindi_enum] -> Bus Creator/256
  [VHAL_LRPindi_enum] -> Bus Creator/255
  [VHAL_RFPindi_enum] -> Bus Creator/254
  [VHAL_LFPindi_enum] -> Bus Creator/253
  [VHAL_RRWheelPSW_raw8] -> Bus Creator/252
  [VHAL_RFWheelPSW_raw8] -> Bus Creator/250
  [VHAL_LFWheelPSW_raw8] -> Bus Creator/249
  [VHAL_RRSensorFail_flg] -> Bus Creator/248
  [VHAL_LRSensorFail_flg] -> Bus Creator/247
  [VHAL_RFSensorFail_flg] -> Bus Creator/246
  [VHAL_LFSensorFail_flg] -> Bus Creator/245
  [VHAL_Flashdatavalid_enum] -> Bus Creator/244
  [VHAL_Flashchkdatavalid_enum] -> Bus Creator/243
  [VHAL_FlashRRID_raw] -> Bus Creator/242
  [VHAL_FlashLRID_raw] -> Bus Creator/241
  [VHAL_FlashRFID_raw] -> Bus Creator/240
  [VHAL_FlashLFID_raw] -> Bus Creator/239
  [VHAL_FlashChkRRID_raw] -> Bus Creator/238
  [VHAL_FlashChkLRID_raw] -> Bus Creator/237
  [VHAL_FlashChkRFID_raw] -> Bus Creator/236
  [VHAL_FlashChkLFID_raw] -> Bus Creator/235
  [VHAL_LRWheelPSW_raw8] -> Bus Creator/251
  [VHAL_FlashHMIKey1Func_enum] -> Bus Creator/278  "VHAL_FlashHMIKey1Func_enum"
  [VHAL_FlashHMIKey2Func_enum] -> Bus Creator/279  "VHAL_FlashHMIKey2Func_enum"
  [VHAL_FlashHMIKey3Func_enum] -> Bus Creator/280  "VHAL_FlashHMIKey3Func_enum"
  [VHAL_FlashHMIKey4Func_enum] -> Bus Creator/281  "VHAL_FlashHMIKey4Func_enum"
  [VHAL_FlashHMIKey5Func_enum] -> Bus Creator/282  "VHAL_FlashHMIKey5Func_enum"
  [VHAL_FlashHMIKey6Func_enum] -> Bus Creator/283  "VHAL_FlashHMIKey6Func_enum"
  [VHAL_FlashHMIKey7Func_enum] -> Bus Creator/284  "VHAL_FlashHMIKey7Func_enum"
  [VHAL_FlashHMIKey8Func_enum] -> Bus Creator/285  "VHAL_FlashHMIKey8Func_enum"
  [VHAL_FlashAutoWipHSpdEN_flg] -> Bus Creator/286  "VHAL_FlashAutoWipHSpdEN_flg"
  [VHAL_FlashDIDModelVersion_raw] -> Bus Creator/287  "VHAL_FlashDIDModelVersion_raw"
  [VHAL_FlashDIDModelVersionChkSum_raw] -> Bus Creator/288  "VHAL_FlashDIDModelVersionChkSum_raw"
  [HAL_NvmReadData_raw] -> Selector2/1
  Selector2/1 -> Demux3/1
  Data Type Conversion300/1 -> [VHAL_FlashAirIntenZone1MSet3_enum]  "VHAL_FlashAirIntenZone1MSet3_enum"
  Data Type Conversion251/1 -> [VHAL_FlashAirIntenZone1MSet2_enum]  "VHAL_FlashAirIntenZone1MSet2_enum"
  Data Type Conversion302/1 -> [VHAL_FlashAirIntenZone1MSet5_enum]  "VHAL_FlashAirIntenZone1MSet5_enum"
  Data Type Conversion301/1 -> [VHAL_FlashAirIntenZone1MSet4_enum]  "VHAL_FlashAirIntenZone1MSet4_enum"
  Data Type Conversion303/1 -> [VHAL_FlashAirIntenZone1MSet7_enum]  "VHAL_FlashAirIntenZone1MSet7_enum"
  Data Type Conversion304/1 -> [VHAL_FlashAirIntenZone3MSet2_enum]  "VHAL_FlashAirIntenZone3MSet2_enum"
  Data Type Conversion305/1 -> [VHAL_FlashAirIntenZone3MSet3_enum]  "VHAL_FlashAirIntenZone3MSet3_enum"
  Data Type Conversion307/1 -> [VHAL_FlashAirIntenZone3MSet5_enum]  "VHAL_FlashAirIntenZone3MSet5_enum"
  Data Type Conversion306/1 -> [VHAL_FlashAirIntenZone3MSet4_enum]  "VHAL_FlashAirIntenZone3MSet4_enum"
  Data Type Conversion308/1 -> [VHAL_FlashAirIntenZone3MSet7_enum]  "VHAL_FlashAirIntenZone3MSet7_enum"
  Data Type Conversion312/1 -> [VHAL_FlashPsEVentModeStaSet457_enum]  "VHAL_FlashPsEVentModeStaSet457_enum"
  Data Type Conversion310/1 -> [VHAL_FlashFGSAirIntStaSet457_enum]  "VHAL_FlashFGSAirIntStaSet457_enum"
  Data Type Conversion311/1 -> [VHAL_FlashDrEVentModeStaSet457_enum]  "VHAL_FlashDrEVentModeStaSet457_enum"
  Data Type Conversion309/1 -> [VHAL_FlashFGSChStaSet457_enum]  "VHAL_FlashFGSChStaSet457_enum"
  Data Type Conversion313/1 -> [VHAL_FlashDrEVentZStaSet2_enum]  "VHAL_FlashDrEVentZStaSet2_enum"
  Data Type Conversion314/1 -> [VHAL_FlashDrEVentZStaSet3_enum]  "VHAL_FlashDrEVentZStaSet3_enum"
  Data Type Conversion316/1 -> [VHAL_FlashDrEVentZStaSet5_enum]  "VHAL_FlashDrEVentZStaSet5_enum"
  Data Type Conversion315/1 -> [VHAL_FlashDrEVentZStaSet4_enum]  "VHAL_FlashDrEVentZStaSet4_enum"
  Data Type Conversion317/1 -> [VHAL_FlashDrEVentZStaSet7_enum]  "VHAL_FlashDrEVentZStaSet7_enum"
  Data Type Conversion318/1 -> [VHAL_FlashCLEVentZStaSet2_enum]  "VHAL_FlashCLEVentZStaSet2_enum"
  Data Type Conversion319/1 -> [VHAL_FlashCLEVentZStaSet3_enum]  "VHAL_FlashCLEVentZStaSet3_enum"
  Data Type Conversion321/1 -> [VHAL_FlashCLEVentZStaSet5_enum]  "VHAL_FlashCLEVentZStaSet5_enum"
  Data Type Conversion320/1 -> [VHAL_FlashCLEVentZStaSet4_enum]  "VHAL_FlashCLEVentZStaSet4_enum"
  Data Type Conversion322/1 -> [VHAL_FlashCLEVentZStaSet7_enum]  "VHAL_FlashCLEVentZStaSet7_enum"
  Data Type Conversion326/1 -> [VHAL_FlashPsEVentZStaSet5_enum]  "VHAL_FlashPsEVentZStaSet5_enum"
  Data Type Conversion325/1 -> [VHAL_FlashPsEVentZStaSet4_enum]  "VHAL_FlashPsEVentZStaSet4_enum"
  Data Type Conversion324/1 -> [VHAL_FlashPsEVentZStaSet3_enum]  "VHAL_FlashPsEVentZStaSet3_enum"
  Data Type Conversion327/1 -> [VHAL_FlashPsEVentZStaSet7_enum]  "VHAL_FlashPsEVentZStaSet7_enum"
  Data Type Conversion323/1 -> [VHAL_FlashPsEVentZStaSet2_enum]  "VHAL_FlashPsEVentZStaSet2_enum"
  Data Type Conversion331/1 -> [VHAL_FlashCREVentZStaSet5_enum]  "VHAL_FlashCREVentZStaSet5_enum"
  Data Type Conversion330/1 -> [VHAL_FlashCREVentZStaSet4_enum]  "VHAL_FlashCREVentZStaSet4_enum"
  Data Type Conversion329/1 -> [VHAL_FlashCREVentZStaSet3_enum]  "VHAL_FlashCREVentZStaSet3_enum"
  Data Type Conversion332/1 -> [VHAL_FlashCREVentZStaSet7_enum]  "VHAL_FlashCREVentZStaSet7_enum"
  Data Type Conversion328/1 -> [VHAL_FlashCREVentZStaSet2_enum]  "VHAL_FlashCREVentZStaSet2_enum"
  Data Type Conversion336/1 -> [VHAL_FlashDrEVentYStaSet5_enum]  "VHAL_FlashDrEVentYStaSet5_enum"
  Data Type Conversion335/1 -> [VHAL_FlashDrEVentYStaSet4_enum]  "VHAL_FlashDrEVentYStaSet4_enum"
  Data Type Conversion334/1 -> [VHAL_FlashDrEVentYStaSet3_enum]  "VHAL_FlashDrEVentYStaSet3_enum"
  Data Type Conversion337/1 -> [VHAL_FlashDrEVentYStaSet7_enum]  "VHAL_FlashDrEVentYStaSet7_enum"
  Data Type Conversion333/1 -> [VHAL_FlashDrEVentYStaSet2_enum]  "VHAL_FlashDrEVentYStaSet2_enum"
  Data Type Conversion341/1 -> [VHAL_FlashCLEVentYStaSet5_enum]  "VHAL_FlashCLEVentYStaSet5_enum"
  Data Type Conversion340/1 -> [VHAL_FlashCLEVentYStaSet4_enum]  "VHAL_FlashCLEVentYStaSet4_enum"
  Data Type Conversion339/1 -> [VHAL_FlashCLEVentYStaSet3_enum]  "VHAL_FlashCLEVentYStaSet3_enum"
  Data Type Conversion342/1 -> [VHAL_FlashCLEVentYStaSet7_enum]  "VHAL_FlashCLEVentYStaSet7_enum"
  Data Type Conversion338/1 -> [VHAL_FlashCLEVentYStaSet2_enum]  "VHAL_FlashCLEVentYStaSet2_enum"
  Data Type Conversion346/1 -> [VHAL_FlashPsEVentYStaSet5_enum]  "VHAL_FlashPsEVentYStaSet5_enum"
  Data Type Conversion345/1 -> [VHAL_FlashPsEVentYStaSet4_enum]  "VHAL_FlashPsEVentYStaSet4_enum"
  Data Type Conversion344/1 -> [VHAL_FlashPsEVentYStaSet3_enum]  "VHAL_FlashPsEVentYStaSet3_enum"
  Data Type Conversion347/1 -> [VHAL_FlashPsEVentYStaSet7_enum]  "VHAL_FlashPsEVentYStaSet7_enum"
  Data Type Conversion343/1 -> [VHAL_FlashPsEVentYStaSet2_enum]  "VHAL_FlashPsEVentYStaSet2_enum"
  Data Type Conversion351/1 -> [VHAL_FlashCREVentYStaSet5_enum]  "VHAL_FlashCREVentYStaSet5_enum"
  Data Type Conversion350/1 -> [VHAL_FlashCREVentYStaSet4_enum]  "VHAL_FlashCREVentYStaSet4_enum"
  Data Type Conversion349/1 -> [VHAL_FlashCREVentYStaSet3_enum]  "VHAL_FlashCREVentYStaSet3_enum"
  Data Type Conversion352/1 -> [VHAL_FlashCREVentYStaSet7_enum]  "VHAL_FlashCREVentYStaSet7_enum"
  Data Type Conversion348/1 -> [VHAL_FlashCREVentYStaSet2_enum]  "VHAL_FlashCREVentYStaSet2_enum"
  Data Type Conversion354/1 -> [VHAL_FlashSettempZon1Set2_enum]  "VHAL_FlashSettempZon1Set2_enum"
  Data Type Conversion353/1 -> [VHAL_FlashACModeSet457_enum]  "VHAL_FlashACModeSet457_enum"
  Data Type Conversion355/1 -> [VHAL_FlashSettempZon1Set3_enum]  "VHAL_FlashSettempZon1Set3_enum"
  Data Type Conversion357/1 -> [VHAL_FlashSettempZon1Set5_enum]  "VHAL_FlashSettempZon1Set5_enum"
  Data Type Conversion356/1 -> [VHAL_FlashSettempZon1Set4_enum]  "VHAL_FlashSettempZon1Set4_enum"
  Data Type Conversion358/1 -> [VHAL_FlashSettempZon1Set7_enum]  "VHAL_FlashSettempZon1Set7_enum"
  Demux3/1 -> Data Type Conversion251/1
  Demux3/2 -> Data Type Conversion300/1
  Demux3/3 -> Data Type Conversion301/1
  Demux3/4 -> Data Type Conversion302/1
  Demux3/5 -> Data Type Conversion303/1
  Demux3/6 -> Data Type Conversion304/1
  Demux3/7 -> Data Type Conversion305/1
  Demux3/8 -> Data Type Conversion306/1
  Demux3/9 -> Data Type Conversion307/1
  Demux3/10 -> Data Type Conversion308/1
  Demux3/11 -> Data Type Conversion309/1
  Demux3/12 -> Data Type Conversion310/1
  Demux3/13 -> Data Type Conversion311/1
  Demux3/14 -> Data Type Conversion312/1
  Demux3/15 -> Data Type Conversion313/1
  Demux3/16 -> Data Type Conversion314/1
  Demux3/17 -> Data Type Conversion315/1
  Demux3/18 -> Data Type Conversion316/1
  Demux3/19 -> Data Type Conversion317/1
  Demux3/20 -> Data Type Conversion318/1
  Demux3/21 -> Data Type Conversion319/1
  Demux3/22 -> Data Type Conversion320/1
  Demux3/23 -> Data Type Conversion321/1
  Demux3/24 -> Data Type Conversion322/1
  Demux3/25 -> Data Type Conversion323/1
  Demux3/26 -> Data Type Conversion324/1
  Demux3/27 -> Data Type Conversion325/1
  Demux3/28 -> Data Type Conversion326/1
  Demux3/29 -> Data Type Conversion327/1
  Demux3/30 -> Data Type Conversion328/1
  Demux3/31 -> Data Type Conversion329/1
  Demux3/32 -> Data Type Conversion330/1
  Demux3/33 -> Data Type Conversion331/1
  Demux3/34 -> Data Type Conversion332/1
  Demux3/35 -> Data Type Conversion333/1
  Demux3/36 -> Data Type Conversion334/1
  Demux3/37 -> Data Type Conversion335/1
  Demux3/38 -> Data Type Conversion336/1
  Demux3/39 -> Data Type Conversion337/1
  Demux3/40 -> Data Type Conversion338/1
  Demux3/41 -> Data Type Conversion339/1
  Demux3/42 -> Data Type Conversion340/1
  Demux3/43 -> Data Type Conversion341/1
  Demux3/44 -> Data Type Conversion342/1
  Demux3/45 -> Data Type Conversion343/1
  Demux3/46 -> Data Type Conversion344/1
  Demux3/47 -> Data Type Conversion345/1
  Demux3/48 -> Data Type Conversion346/1
  Demux3/49 -> Data Type Conversion347/1
  Demux3/50 -> Data Type Conversion348/1
  Demux3/51 -> Data Type Conversion349/1
  Demux3/52 -> Data Type Conversion350/1
  Demux3/53 -> Data Type Conversion351/1
  Demux3/54 -> Data Type Conversion352/1
  Demux3/55 -> Data Type Conversion353/1
  Demux3/56 -> Data Type Conversion354/1
  Demux3/57 -> Data Type Conversion355/1
  Demux3/58 -> Data Type Conversion356/1
  Demux3/59 -> Data Type Conversion357/1
  Demux3/60 -> Data Type Conversion358/1
  [VHAL_FlashAirIntenZone1MSet2_enum] -> Bus Creator/289
  [VHAL_FlashAirIntenZone1MSet3_enum] -> Bus Creator/290
  [VHAL_FlashAirIntenZone1MSet4_enum] -> Bus Creator/291
  [VHAL_FlashAirIntenZone1MSet5_enum] -> Bus Creator/292
  [VHAL_FlashAirIntenZone1MSet7_enum] -> Bus Creator/293
  [VHAL_FlashAirIntenZone3MSet2_enum] -> Bus Creator/294
  [VHAL_FlashAirIntenZone3MSet3_enum] -> Bus Creator/295
  [VHAL_FlashAirIntenZone3MSet4_enum] -> Bus Creator/296
  [VHAL_FlashAirIntenZone3MSet5_enum] -> Bus Creator/297
  [VHAL_FlashAirIntenZone3MSet7_enum] -> Bus Creator/298
  [VHAL_FlashFGSChStaSet457_enum] -> Bus Creator/299
  [VHAL_FlashFGSAirIntStaSet457_enum] -> Bus Creator/300
  [VHAL_FlashDrEVentModeStaSet457_enum] -> Bus Creator/301
  [VHAL_FlashPsEVentModeStaSet457_enum] -> Bus Creator/302
  [VHAL_FlashDrEVentZStaSet2_enum] -> Bus Creator/303
  [VHAL_FlashDrEVentZStaSet3_enum] -> Bus Creator/304
  [VHAL_FlashDrEVentZStaSet4_enum] -> Bus Creator/305
  [VHAL_FlashDrEVentZStaSet5_enum] -> Bus Creator/306
  [VHAL_FlashDrEVentZStaSet7_enum] -> Bus Creator/307
  [VHAL_FlashCLEVentZStaSet2_enum] -> Bus Creator/308
  [VHAL_FlashCLEVentZStaSet3_enum] -> Bus Creator/309
  [VHAL_FlashCLEVentZStaSet4_enum] -> Bus Creator/310
  [VHAL_FlashCLEVentZStaSet5_enum] -> Bus Creator/311
  [VHAL_FlashCLEVentZStaSet7_enum] -> Bus Creator/312
  [VHAL_FlashPsEVentZStaSet2_enum] -> Bus Creator/313
  [VHAL_FlashPsEVentZStaSet3_enum] -> Bus Creator/314
  [VHAL_FlashPsEVentZStaSet4_enum] -> Bus Creator/315
  [VHAL_FlashPsEVentZStaSet5_enum] -> Bus Creator/316
  [VHAL_FlashPsEVentZStaSet7_enum] -> Bus Creator/317
  [VHAL_FlashCREVentZStaSet2_enum] -> Bus Creator/318
  [VHAL_FlashCREVentZStaSet3_enum] -> Bus Creator/319
  [VHAL_FlashCREVentZStaSet4_enum] -> Bus Creator/320
  [VHAL_FlashCREVentZStaSet5_enum] -> Bus Creator/321
  [VHAL_FlashCREVentZStaSet7_enum] -> Bus Creator/322
  [VHAL_FlashDrEVentYStaSet2_enum] -> Bus Creator/323
  [VHAL_FlashDrEVentYStaSet3_enum] -> Bus Creator/324
  [VHAL_FlashDrEVentYStaSet4_enum] -> Bus Creator/325
  [VHAL_FlashDrEVentYStaSet5_enum] -> Bus Creator/326
  [VHAL_FlashDrEVentYStaSet7_enum] -> Bus Creator/327
  [VHAL_FlashCLEVentYStaSet2_enum] -> Bus Creator/328
  [VHAL_FlashCLEVentYStaSet3_enum] -> Bus Creator/329
  [VHAL_FlashCLEVentYStaSet4_enum] -> Bus Creator/330
  [VHAL_FlashCLEVentYStaSet5_enum] -> Bus Creator/331
  [VHAL_FlashCLEVentYStaSet7_enum] -> Bus Creator/332
  [VHAL_FlashPsEVentYStaSet2_enum] -> Bus Creator/333
  [VHAL_FlashPsEVentYStaSet3_enum] -> Bus Creator/334
  [VHAL_FlashPsEVentYStaSet4_enum] -> Bus Creator/335
  [VHAL_FlashPsEVentYStaSet5_enum] -> Bus Creator/336
  [VHAL_FlashPsEVentYStaSet7_enum] -> Bus Creator/337
  [VHAL_FlashCREVentYStaSet2_enum] -> Bus Creator/338
  [VHAL_FlashCREVentYStaSet3_enum] -> Bus Creator/339
  [VHAL_FlashCREVentYStaSet4_enum] -> Bus Creator/340
  [VHAL_FlashCREVentYStaSet5_enum] -> Bus Creator/341
  [VHAL_FlashCREVentYStaSet7_enum] -> Bus Creator/342
  [VHAL_FlashACModeSet457_enum] -> Bus Creator/343
  [VHAL_FlashSettempZon1Set2_enum] -> Bus Creator/344
  [VHAL_FlashSettempZon1Set3_enum] -> Bus Creator/345
  [VHAL_FlashSettempZon1Set7_enum] -> Bus Creator/348
  [VHAL_FlashSettempZon1Set4_enum] -> Bus Creator/346
  [VHAL_FlashSettempZon1Set5_enum] -> Bus Creator/347
  Data Type Conversion359/1 -> [VHAL_FlashJugKeepUnLZone_flg]  "VHAL_FlashJugKeepUnLZone_flg"
  Demux3/61 -> Data Type Conversion359/1
  [VHAL_FlashJugKeepUnLZone_flg] -> Bus Creator/349
  Data Type Conversion360/1 -> Bus Creator/17  "VHAL_DrivingMode_cnt"
  Data Type Conversion361/1 -> Bus Creator/18  "VHAL_ModelYear_cnt"
  Data Type Conversion362/1 -> Bus Creator/19  "VHAL_Var4_cnt"
  Data Type Conversion363/1 -> Bus Creator/20  "VHAL_Var5_cnt"
  Demux/32 -> Data Type Conversion28/1
  Demux/31 -> Data Type Conversion27/1
  Demux/30 -> Data Type Conversion26/1
  Demux/29 -> Data Type Conversion25/1
  Demux/28 -> Data Type Conversion24/1
  Demux/27 -> Data Type Conversion23/1
  Demux/26 -> Data Type Conversion22/1
  Demux/25 -> Data Type Conversion21/1
  Demux/24 -> Data Type Conversion20/1
  Demux/23 -> Data Type Conversion19/1
  Demux/22 -> Data Type Conversion18/1
  Demux/21 -> Data Type Conversion17/1
  Demux/20 -> Data Type Conversion363/1
  Demux/19 -> Data Type Conversion362/1
  Demux/18 -> Data Type Conversion361/1
  Demux/17 -> Data Type Conversion360/1
  Demux/33 -> Terminator3/1
